simulink library "pneAux_rebuild_generic_std"  (R2016a)
settings: Solver=VariableStepAuto  StartTime=0.0  StopTime=10.0  RelTol=1e-3
undefined symbols (not defined in the file): sMP
(part 2 of 2)

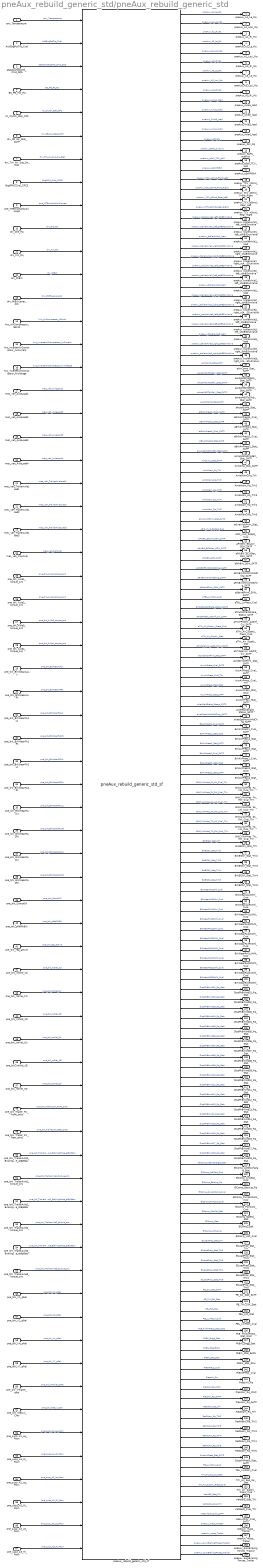
== system pneAux_rebuild_generic_std/pneAux_rebuild_generic_std ==
  env_Temperature : Inport
  ActlEngPctTrq_Cval : Inport  Port=2
  aSatpAutoOpMd_Cmd_SDS : Inport  Port=3
  BS_PB_Fct_Rq : Inport  Port=4
  ch_Clutch_Stat_CPC : Inport  Port=5
  drv_PB_Sw_Stat_SATP : Inport  Port=6
  drv_Trlr_Air_Sup_Sw_Stat : Inport  Port=7
  EngRPM_Cval_CPC3 : Inport  Port=8
  pne_MTBmodusSwAllowed : Inport  Port=9
  drv_DrS_Rq : Inport  Port=10
  drv_Knl_Rq : Inport  Port=11
  drv_PkBrk : Inport  Port=12
  drv_PkBrkLever_pos : Inport  Port=13
  hvs_AirCompressor_nEmot : Inport  Port=14
  hvs_InverterAirCompressor_hvCurrent : Inport  Port=15
  hvs_InverterAirCompressor_hvVoltage : Inport  Port=16
  mec_veh_AxleLoad1 : Inport  Port=17
  mec_veh_AxleLoad2 : Inport  Port=18
  mec_veh_AxleLoad3 : Inport  Port=19
  mec_veh_AxleLoad4 : Inport  Port=20
  mec_veh_TrailerAxleLoad1 : Inport  Port=21
  mec_veh_TrailerAxleLoad2 : Inport  Port=22
  mec_veh_TrailerAxleLoad3 : Inport  Port=23
  mec_veh_transVel : Inport  Port=24
  pne_brk_Axle1_torque_sns : Inport  Port=25
  pne_brk_Axle2_torque_sns : Inport  Port=26
  pne_brk_Axle3_torque_sns : Inport  Port=27
  pne_brk_Axle4_torque_sns : Inport  Port=28
  pne_brk_BrkWearAALt : Inport  Port=29
  pne_brk_BrkWearAARt : Inport  Port=30
  pne_brk_BrkWearFA1Lt : Inport  Port=31
  pne_brk_BrkWearFA1Rt : Inport  Port=32
  pne_brk_BrkWearFA2Lt : Inport  Port=33
  pne_brk_BrkWearFA2Rt : Inport  Port=34
  pne_brk_BrkWearRA1Lt : Inport  Port=35
  pne_brk_BrkWearRA1Rt : Inport  Port=36
  pne_brk_BrkWearRA2Lt : Inport  Port=37
  pne_brk_BrkWearRA2Rt : Inport  Port=38
  pne_brk_CompON : Inport  Port=39
  pne_brk_pRelPkBrk : Inport  Port=40
  pne_brk_reg_active : Inport  Port=41
  pne_brk_rotVel_t1l : Inport  Port=42
  pne_brk_rotVel_t1r : Inport  Port=43
  pne_brk_rotVel_t2l : Inport  Port=44
  pne_brk_rotVel_t2r : Inport  Port=45
  pne_brk_rotVel_t3l : Inport  Port=46
  pne_brk_rotVel_t3r : Inport  Port=47
  pne_brk_Trailer_RV_Front_pAct : Inport  Port=48
  pne_brk_Trailer_RV_Rear_pAct : Inport  Port=49
  pne_brk_TrailerAxle1_BrakingForce_at8p5bar : Inport  Port=50
  pne_brk_TrailerAxle1_torque_sns : Inport  Port=51
  pne_brk_TrailerAxle2_BrakingForce_at8p5bar : Inport  Port=52
  pne_brk_TrailerAxle2_torque_sns : Inport  Port=53
  pne_brk_TrailerAxle3_BrakingForce_at8p5bar : Inport  Port=54
  pne_brk_TrailerAxle3_torque_sns : Inport  Port=55
  pne_brk_V1_pRel : Inport  Port=56
  pne_brk_V2_pRel : Inport  Port=57
  pne_brk_V4_pRel : Inport  Port=58
  pne_brk_V7_pRel : Inport  Port=59
  pne_brk_VTrailer_pRel : Inport  Port=60
  pne_brk_WetLvl_Cntr : Inport  Port=61
  pne_susp_A1_Le_Posn : Inport  Port=62
  pne_susp_A1_Ri_Posn : Inport  Port=63
  pne_susp_A2_Le_Posn : Inport  Port=64
  pne_susp_A2_Ri_Posn : Inport  Port=65
  pne_susp_A3_Le_Posn : Inport  Port=66
  pne_susp_A3_Ri_Posn : Inport  Port=67
  pneAux_rebuild_generic_std_sf : S-Function  FunctionName=pneAux_rebuild_generic_std_sf  Parameters=s1 s2 p1 p2 p3 p4 p5 p6 p7 p8 p9 p10 p11 p12 p13 p14 p15 p16 p17 p18 p19 p20 p21 p22 p23 p24 p25 p26 p27 p28 p29 p30 p31 p32 p33 p34 p35 p36 p37 p38 p39 p40 p41 p42 p43 p44 p45 p46 p47 p48 p49 p50 p51 p52 p53 p54 p55 p56 p57 p58 p59 p60 p61 p62 p63 p64 p65 p66 p67 p68 p69 p70 p71 p72 p73 p74 p75 p76 p77 p78 p79 p80 p81 p82 p83 p84 p85 p86 p87 p88 p89 p90 p91 p92 p93 p94 p95 p96 p97 p98 p99 p100 p101 p102 p103 p104 p105 p106 p107 p108 p109 p110 p111 p112 p113 p114 p115 p116 p117 p118 p119 p120 p121 p122 p123 p124 p125 p126 p127 p128 p129 p130 p131 p132 p133 p134 p135 p136 p137 p138 p139 p140 p141 p142 p143 p144 p145 p146 p147 p148 p149 p150 p151 p152 p153 p154 p155 p156 p157 p158 p159 p160 p161 p162 p163 p164 p165 p166 p167 p168 p169 p170 p171 p172 p173 p174 p175 p176 p177 p178 p179 p180 p181 p182 p183 p184 p185 p186 p187 p188 p189 p190 p191 p192 p193 p194 p195 p196 p197 p198 p199 p200 p201 p202 p203 p204 p205 p206 p207 p208 p209 p210 p211 p212 p213 p214 p215 p216 p217 p218 p219 p220 p221 p222 p223 p224 p225 p226 p227 p228 p229 p230 p231 p232 p233 p234 p235 p236 p237 p238 p239 p240 p241 p242 p243 p244 p245 p246 p247 p248 p249 p250 p251 p252 p253 p254 p255 p256 p257  SFunctionModules=<binary blob, 526 chars, not shown>  SFunctionDeploymentMode=off  EnableBusSupport=off  mask{s1=s1, s2=s2, initCmd='Parameters_pneAux_rebuild_generic_std_sf', p1=p1, p2=p2, p3=p3, p4=p4, p5=p5, p6=p6, p7=p7, p8=p8, p9=p9, p10=p10, p11=p11, p12=p12, p13=p13, p14=p14, p15=p15, p16=p16, p17=p17, p18=p18, p19=p19, p20=p20, p21=p21, p22=p22, p23=p23, p24=p24, p25=p25, p26=p26, p27=p27, p28=p28, p29=p29, p30=p30, p31=p31, p32=p32, p33=p33, p34=p34, p35=p35, p36=p36, p37=p37, p38=p38, p39=p39, p40=p40, p41=p41, p42=p42, p43=p43, p44=p44, p45=p45, p46=p46, p47=p47, p48=p48, p49=p49, p50=p50, p51=p51, p52=p52, p53=p53, p54=p54, p55=p55, p56=p56, p57=p57, p58=p58, p59=p59, p60=p60, p61=p61, p62=p62, p63=p63, p64=p64, p65=p65, p66=p66, p67=p67, p68=p68, p69=p69, p70=p70, p71=p71, p72=p72, p73=p73, p74=p74, p75=p75, p76=p76, p77=p77, p78=p78, p79=p79, p80=p80, p81=p81, p82=p82, p83=p83, p84=p84, p85=p85, p86=p86, p87=p87, p88=p88, p89=p89, p90=p90, p91=p91, p92=p92, p93=p93, p94=p94, p95=p95, p96=p96, p97=p97, p98=p98, p99=p99, p100=p100, p101=p101, p102=p102, p103=p103, p104=p104, p105=p105, p106=p106, p107=p107, p108=p108, p109=p109, p110=p110, p111=p111, p112=p112, p113=p113, p114=p114, p115=p115, p116=p116, p117=p117, p118=p118, p119=p119, p120=p120, p121=p121, p122=p122, p123=p123, p124=p124, p125=p125, p126=p126, p127=p127, p128=p128, p129=p129, p130=p130, p131=p131, p132=p132, p133=p133, p134=p134, p135=p135, p136=p136, p137=p137, p138=p138, p139=p139, p140=p140, p141=p141, p142=p142, p143=p143, p144=p144, p145=p145, p146=p146, p147=p147, p148=p148, p149=p149, p150=p150, p151=p151, p152=p152, p153=p153, p154=p154, p155=p155, p156=p156, p157=p157, p158=p158, p159=p159, p160=p160, p161=p161, p162=p162, p163=p163, p164=p164, p165=p165, p166=p166, p167=p167, p168=p168, p169=p169, p170=p170, p171=p171, p172=p172, p173=p173, p174=p174, p175=p175, p176=p176, p177=p177, p178=p178, p179=p179, p180=p180, p181=p181, p182=p182, p183=p183, p184=p184, p185=p185, p186=p186, p187=p187, p188=p188, p189=p189, p190=p190, p191=p191, p192=p192, p193=p193, p194=p194, p195=p195, p196=p196, p197=p197, p198=p198, p199=p199, p200=p200, p201=p201, p202=p202, p203=p203, p204=p204, p205=p205, p206=p206, p207=p207, p208=p208, p209=p209, p210=p210, p211=p211, p212=p212, p213=p213, p214=p214, p215=p215, p216=p216, p217=p217, p218=p218, p219=p219, p220=p220, p221=p221, p222=p222, p223=p223, p224=p224, p225=p225, p226=p226, p227=p227, p228=p228, p229=p229, p230=p230, p231=p231, p232=p232, p233=p233, p234=p234, p235=p235, p236=p236, p237=p237, p238=p238, p239=p239, p240=p240, p241=p241, p242=p242, p243=p243, p244=p244, p245=p245, p246=p246, p247=p247, p248=p248, p249=p249, p250=p250, p251=p251, p252=p252, p253=p253, p254=p254, p255=p255, p256=p256, p257=p257}
      mask prompts: s1 "Solver Type: settings_iMode [-]"; s2 "Solver Step Size: settings_dt [s]"; initCmd "Initialization command"; p1 "aAirComp_Stat_SATP, Compressor status: 0,1,2,3 / inactiv, active, err, SNA export=true name=aAirComp_Stat_SATP prio=1 dataSetName=std dataClassType=initIO dataClassName=initIO unit='-' description='Compressor status: 0,1,2,3 / inactiv, active, err, SNA': pneAux.aAirComp_Stat_SATP_0 [-]"; p2 "aAutoMd1To2Rdy_Stat_SATP, L4 - Driver mode: 0,1,2,3 / not ready, ready, reserved, SNA ((ATG) Readiness status of SATP to transition from mode 1 to mode 2) export=true name=aAutoMd1To2Rdy_Stat_SATP prio=1 dataSetName=std dataClassType=initIO dataClassName=initIO unit='-' description='L4 - Driver mode: 0,1,2,3 / not ready, ready, reserved, SNA ((ATG) Readiness status of SATP to transition from mode 1 to mode 2)': pneAux.aAutoMd1To2Rdy_Stat_SATP_0 [-]"; p3 "aAutoMd1To3Rdy_Stat_SATP, L4 - Driver mode: 0,1,2,3 / not ready, ready, reserved, SNA ((ATG) Readiness status of SATP to transition from mode 1 to mode 3) export=true name=aAutoMd1To3Rdy_Stat_SATP prio=1 dataSetName=std dataClassType=initIO dataClassName=initIO unit='-' description='L4 - Driver mode: 0,1,2,3 / not ready, ready, reserved, SNA ((ATG) Readiness status of SATP to transition from mode 1 to mode 3)': pneAux.aAutoMd1To3Rdy_Stat_SATP_0 [-]"; p4 "aAutoMd3To1Rdy_Stat_SATP, L4 - Driver mode: 0,1,2,3 / not ready, ready, reserved, SNA ((ATG) Readiness status of SATP to transition from mode 3 to mode 1) export=true name=aAutoMd3To1Rdy_Stat_SATP prio=1 dataSetName=std dataClassType=initIO dataClassName=initIO unit='-' description='L4 - Driver mode: 0,1,2,3 / not ready, ready, reserved, SNA ((ATG) Readiness status of SATP to transition from mode 3 to mode 1)': pneAux.aAutoMd3To1Rdy_Stat_SATP_0 [-]"; p5 "aAutoOpMd_Stat_SATP, 0,1,2,3 /  MODE_1 Manual Mode, L4_IFTD SAE L4 with IFTD, L4_NDC SAE L4 with no driver controls, SNA Signal not Available export=true name=aAutoOpMd_Stat_SATP prio=1 dataSetName=std dataClassType=initIO dataClassName=initIO unit='-' description='0,1,2,3 /  MODE_1 Manual Mode, L4_IFTD SAE L4 with IFTD, L4_NDC SAE L4 with no driver controls, SNA Signal not Available': pneAux.aAutoOpMd_Stat_SATP_0 [-]"; p6 "aBrkAirPress1_Cval_SATP (init) export=true name=aBrkAirPress1_Cval_SATP prio=1 dataSetName=std dataClassType=initIO dataClassName=initIO unit=kPa description='aBrkAirPress1_Cval_SATP': pneAux.aBrkAirPress1_Cval_SATP_0 [-]"; p7 "aBrkAirPress1_Stat_SATP (init) export=true name=aBrkAirPress1_Stat_SATP prio=1 dataSetName=std dataClassType=initIO dataClassName=initIO unit=kPa description='aBrkAirPress1_Stat_SATP': pneAux.aBrkAirPress1_Stat_SATP_0 [-]"; p8 "aBrkAirPress2_Cval_SATP (init) export=true name=aBrkAirPress2_Cval_SATP prio=1 dataSetName=std dataClassType=initIO dataClassName=initIO unit=kPa description='aBrkAirPress2_Cval_SATP': pneAux.aBrkAirPress2_Cval_SATP_0 [-]"; p9 "aBrkAirPress2_Stat_SATP (init) export=true name=aBrkAirPress2_Stat_SATP prio=1 dataSetName=std dataClassType=initIO dataClassName=initIO unit=kPa description='aBrkAirPress2_Stat_SATP': pneAux.aBrkAirPress2_Stat_SATP_0 [-]"; p10 "ActlEngPctTrq_Cval (init) export=true name=ActlEngPctTrq_Cval prio=1 dataSetName=std dataClassType=initIO dataClassName=initIO unit='-' description='ActlEngPctTrq_Cval': pneAux.ActlEngPctTrq_Cval_0 [-]"; p11 "aImplsblMdCmdErr_Stat_SATP, 0,1,2,3 /  OK, invalid, reserved, SNA export=true name=aImplsblMdCmdErr_Stat_SATP prio=1 dataSetName=std dataClassType=initIO dataClassName=initIO unit='-' description='0,1,2,3 /  OK, invalid, reserved, SNA': pneAux.aImplsblMdCmdErr_Stat_SATP_0 [-]"; p12 "AirComp_Stat_SATP, Compressor status: 0,1,2,3 / inactiv, active, err, SNA export=true name=AirComp_Stat_SATP prio=1 dataSetName=std dataClassType=initIO dataClassName=initIO unit='-' description='Compressor status: 0,1,2,3 / inactiv, active, err, SNA': pneAux.AirComp_Stat_SATP_0 [-]"; p13 "AmbWarn_Rq_Trlr2,   export=true name=AmbWarn_Rq_Trlr2 prio=1 dataSetName=std dataClassType=initIO dataClassName=initIO unit='-' description=' ': pneAux.AmbWarn_Rq_Trlr2_0 [-]"; p14 "AmbWarn_Rq_Trlr3,   export=true name=AmbWarn_Rq_Trlr3 prio=1 dataSetName=std dataClassType=initIO dataClassName=initIO unit='-' description=' ': pneAux.AmbWarn_Rq_Trlr3_0 [-]"; p15 "AmbWarn_Rq_Trlr4,   export=true name=AmbWarn_Rq_Trlr4 prio=1 dataSetName=std dataClassType=initIO dataClassName=initIO unit='-' description=' ': pneAux.AmbWarn_Rq_Trlr4_0 [-]"; p16 "AmbWarn_Rq_Trlr5,   export=true name=AmbWarn_Rq_Trlr5 prio=1 dataSetName=std dataClassType=initIO dataClassName=initIO unit='-' description=' ': pneAux.AmbWarn_Rq_Trlr5_0 [-]"; p17 "AmbWarn_Rq_Trlr export=true name=AmbWarn_Rq_Trlr prio=1 dataSetName=std dataClassType=initIO dataClassName=initIO unit='-' description='AmbWarn_Rq_Trlr': pneAux.AmbWarn_Rq_Trlr_0 [-]"; p18 "aOverVoltPrim_Stat_SATP, 0,1,2,3 /  OK, overvoltage, reserved, SNA export=true name=aOverVoltPrim_Stat_SATP prio=1 dataSetName=std dataClassType=initIO dataClassName=initIO unit='-' description='0,1,2,3 /  OK, overvoltage, reserved, SNA': pneAux.aOverVoltPrim_Stat_SATP_0 [-]"; p19 "Inverter 2 Requested Speed API2 for air compressor (init) export=true name=API2_Inv2_RqSpd_Cval prio=1 dataSetName=std dataClassType=initIO dataClassName=initIO unit='-' description='Inverter 2 Requested Speed API2 for air compressor (init)': pneAux.API2_Inv2_RqSpd_Cval_0 [-]"; p20 "aPrkBrk_ECUAir_SOH_SATP,  (ATG) ECU  Air management health status: 0 Fully Operational / 1 Partly Operational / 2 Not Operational / 3 SNA export=true name=aPrkBrk_ECUAir_SOH_SATP prio=1 dataSetName=std dataClassType=initIO dataClassName=initIO unit='-' description=' (ATG) ECU  Air management health status: 0 Fully Operational / 1 Partly Operational / 2 Not Operational / 3 SNA': pneAux.aPrkBrk_ECUAir_SOH_SATP_0 [-]"; p21 "aPrkBrk_ECUGen_SOH_SATP,  (ATG) ECU general health status: 0 Fully Operational / 1 Partly Operational / 2 Not Operational / 3 SNA export=true name=aPrkBrk_ECUGen_SOH_SATP prio=1 dataSetName=std dataClassType=initIO dataClassName=initIO unit='-' description=' (ATG) ECU general health status: 0 Fully Operational / 1 Partly Operational / 2 Not Operational / 3 SNA': pneAux.aPrkBrk_ECUGen_SOH_SATP_0 [-]"; p22 "aPrkBrk_SOH_SATP,  (ATG) Parking Brake System Health Status: 0 Fully Operational / 1 Partly Operational / 2 Not Operational / 3 SNA export=true name=aPrkBrk_SOH_SATP prio=1 dataSetName=std dataClassType=initIO dataClassName=initIO unit='-' description=' (ATG) Parking Brake System Health Status: 0 Fully Operational / 1 Partly Operational / 2 Not Operational / 3 SNA': pneAux.aPrkBrk_SOH_SATP_0 [-]"; p23 "aPrkBrkFltIntrlckMdChng_SATP, 0,1,2,3 /  NoT met, met, reserved, SNA ((ATG) Current status in SATP for the Fault interlock for mode change) export=true name=aPrkBrkFltIntrlckMdChng_SATP prio=1 dataSetName=std dataClassType=initIO dataClassName=initIO unit='-' description='0,1,2,3 /  NoT met, met, reserved, SNA ((ATG) Current status in SATP for the Fault interlock for mode change)': pneAux.aPrkBrkFltIntrlckMdChng_SATP_0 [-]"; p24 "aPrkBrkIntrlckMdChng_SATP, 0,1,2,3 /  NoT met, met, reserved, SNA ((ATG) Current status in SATP for the park brake interlock for mode change) export=true name=aPrkBrkIntrlckMdChng_SATP prio=1 dataSetName=std dataClassType=initIO dataClassName=initIO unit='-' description='0,1,2,3 /  NoT met, met, reserved, SNA ((ATG) Current status in SATP for the park brake interlock for mode change)': pneAux.aPrkBrkIntrlckMdChng_SATP_0 [-]"; p25 "aSatpAutoOpMd_Cmd_SDS (init) export=true name=aSatpAutoOpMd_Cmd_SDS prio=1 dataSetName=std dataClassType=initIO dataClassName=initIO unit='-' description='SATP operational mode command by SDS': pneAux.aSatpAutoOpMd_Cmd_SDS_0 [-]"; p26 "aSdsIntfPrim_SOH_SATP,   export=true name=aSdsIntfPrim_SOH_SATP prio=1 dataSetName=std dataClassType=initIO dataClassName=initIO unit='-' description=' ': pneAux.aSdsIntfPrim_SOH_SATP_0 [-]"; p27 "aTBL_LvrPosn_Cval, Lever: 0..100, 101..253,254,255 / 0..100, RES,ERR,SNA export=true name=aTBL_LvrPosn_Cval prio=1 dataSetName=std dataClassType=initIO dataClassName=initIO unit='%' description='Lever: 0..100, 101..253,254,255 / 0..100, RES,ERR,SNA': pneAux.aTBL_LvrPosn_Cval_0 [-]"; p28 "ATBVehicleParameter (0-disabled, 1-enabled) export=true name=ATBVehicleParameter prio=1 dataSetName=pneAux_dummy dataClassType=main dataClassName=main unit='-' description='ATBVehicleParameter (0-disabled, 1-enabled)': pneAux.ATBVehicleParameter [-]"; p29 "aTractorParkBrake_Status_SATP, 0,1,2,6,7 / ENGG Engaged, INT Intermediate Position, DISENGG Disengaged, ERR, SNA ((ATG)  export=true name=aTractorParkBrake_Status_SATP prio=1 dataSetName=std dataClassType=initIO dataClassName=initIO unit='-' description='0,1,2,6,7 / ENGG Engaged, INT Intermediate Position, DISENGG Disengaged, ERR, SNA ((ATG) ': pneAux.aTractorParkBrake_Status_SATP_0 [-]"; p30 "aTrctrPrkBrk_AddInf_Cvl_SATP, 0,1,2,6,7 / DEFLATED Deflated (parked), INT Intermediate, INFLATED Inflated (unparked), ERR, SNA ((ATG)  export=true name=aTrctrPrkBrk_AddInf_Cvl_SATP prio=1 dataSetName=std dataClassType=initIO dataClassName=initIO unit='-' description='0,1,2,6,7 / DEFLATED Deflated (parked), INT Intermediate, INFLATED Inflated (unparked), ERR, SNA ((ATG) ': pneAux.aTrctrPrkBrk_AddInf_Cvl_SATP_0 [-]"; p31 "aTrlr_Air_Supply_Press_Cval, 0..250,251..253,254,255 / 0..2000, RES,ERR,SNA export=true name=aTrlr_Air_Supply_Press_Cval prio=1 dataSetName=std dataClassType=initIO dataClassName=initIO unit='kPa' description='0..250,251..253,254,255 / 0..2000, RES,ERR,SNA': pneAux.aTrlr_Air_Supply_Press_Cval_0 [-]"; p32 "aTrlr_Air_Supply_Stat (init), 0,1,2,3 / SPL supplied, NSPL not supplied, ERR, SAN ((ATG) Trailer Air Supply Current state) export=true name=aTrlr_Air_Supply_Stat prio=1 dataSetName=std dataClassType=initIO dataClassName=initIO unit='-' description='0,1,2,3 / SPL supplied, NSPL not supplied, ERR, SAN ((ATG) Trailer Air Supply Current state)': pneAux.aTrlr_Air_Supply_Stat_0 [-]"; p33 "aTrlrSpplyLn_AddInf_Cvl_SATP, 0,1,2,3 / HIGH_INT Signal integrity High, 1 LOW_INT Signal Integrity low, 2 NO_SENSING no sensing possible, SNA ((ATG) Trailer Supply Line Additional  export=true name=aTrlrSpplyLn_AddInf_Cvl_SATP prio=1 dataSetName=std dataClassType=initIO dataClassName=initIO unit='-' description='0,1,2,3 / HIGH_INT Signal integrity High, 1 LOW_INT Signal Integrity low, 2 NO_SENSING no sensing possible, SNA ((ATG) Trailer Supply Line Additional ': pneAux.aTrlrSpplyLn_AddInf_Cvl_SATP_0 [-]"; p34 "aUnderVoltPrim_Stat_SATP, (ATG) Primary Under Voltage Status SBSP export=true name=aUnderVoltPrim_Stat_SATP prio=1 dataSetName=std dataClassType=initIO dataClassName=initIO unit='-' description='(ATG) Primary Under Voltage Status SBSP': pneAux.aUnderVoltPrim_Stat_SATP_0 [-]"; p35 "AuxAirPress_Cval_SATP (init) export=true name=AuxAirPress_Cval_SATP prio=1 dataSetName=std dataClassType=initIO dataClassName=initIO unit=kPa description='AuxAirPress_Cval_SATP': pneAux.AuxAirPress_Cval_SATP_0 [-]"; p36 "AuxAirPress_Cval_Trlr (init) export=true name=AuxAirPress_Cval_Trlr prio=1 dataSetName=std dataClassType=initIO dataClassName=initIO unit=kPa description='AuxAirPress_Cval_Trlr': pneAux.AuxAirPress_Cval_Trlr_0 [-]"; p37 "AuxAirPress_Stat_ICUC (init) export=true name=AuxAirPress_Stat_ICUC prio=1 dataSetName=std dataClassType=initIO dataClassName=initIO unit=kPa description='AuxAirPress_Stat_ICUC': pneAux.AuxAirPress_Stat_ICUC_0 [-]"; p38 "AuxAirPress_Stat_SATP (init) export=true name=AuxAirPress_Stat_SATP prio=1 dataSetName=std dataClassType=initIO dataClassName=initIO unit=kPa description='AuxAirPress_Stat_SATP': pneAux.AuxAirPress_Stat_SATP_0 [-]"; p39 "aVehParkBrake_Status_SATP, Parking Brake Status entire vehicle: 0,1,2,3,6,7 / SAFE_PARK Safety Parked, NO_DRIVEOFF Drive-Off Inhibited, SAFE_DRIVEOFF_CBN Safe Drive-Off Combined, SAFE_DRIVEOFF_BT Safe Drive-Off- Bobtail, ERR, SNA ((ATG)  export=true name=aVehParkBrake_Status_SATP prio=1 dataSetName=std dataClassType=initIO dataClassName=initIO unit='-' description='Parking Brake Status entire vehicle: 0,1,2,3,6,7 / SAFE_PARK Safety Parked, NO_DRIVEOFF Drive-Off Inhibited, SAFE_DRIVEOFF_CBN Safe Drive-Off Combined, SAFE_DRIVEOFF_BT Safe Drive-Off- Bobtail, ERR, SNA ((ATG) ': pneAux.aVehParkBrake_Status_SATP_0 [-]"; p40 "aVehSpdIntrlckMdChng_SATP, 0,1,2,3 / NoT met, met, reserved, SNA ((ATG) Current status in SATP for the vehicle speed interlock for mode change export=true name=aVehSpdIntrlckMdChng_SATP prio=1 dataSetName=std dataClassType=initIO dataClassName=initIO unit='-' description='0,1,2,3 / NoT met, met, reserved, SNA ((ATG) Current status in SATP for the vehicle speed interlock for mode change': pneAux.aVehSpdIntrlckMdChng_SATP_0 [-]"; p41 "BrkAirPress1_Cval_SATP (init) export=true name=BrkAirPress1_Cval_SATP prio=1 dataSetName=std dataClassType=initIO dataClassName=initIO unit=kPa description='BrkAirPress1_Cval_SATP': pneAux.BrkAirPress1_Cval_SATP_0 [-]"; p42 "BrkAirPress1_Stat_ICUC (init) export=true name=BrkAirPress1_Stat_ICUC prio=1 dataSetName=std dataClassType=initIO dataClassName=initIO unit=kPa description='BrkAirPress1_Stat_ICUC': pneAux.BrkAirPress1_Stat_ICUC_0 [-]"; p43 "BrkAirPress1_Stat_SATP (init) export=true name=BrkAirPress1_Stat_SATP prio=1 dataSetName=std dataClassType=initIO dataClassName=initIO unit=kPa description='BrkAirPress1_Stat_SATP': pneAux.BrkAirPress1_Stat_SATP_0 [-]"; p44 "BrkAirPress2_Cval_SATP (init) export=true name=BrkAirPress2_Cval_SATP prio=1 dataSetName=std dataClassType=initIO dataClassName=initIO unit=kPa description='BrkAirPress2_Cval_SATP': pneAux.BrkAirPress2_Cval_SATP_0 [-]"; p45 "BrkAirPress2_Stat_ICUC (init) export=true name=BrkAirPress2_Stat_ICUC prio=1 dataSetName=std dataClassType=initIO dataClassName=initIO unit=kPa description='BrkAirPress2_Stat_ICUC': pneAux.BrkAirPress2_Stat_ICUC_0 [-]"; p46 "BrkAirPress2_Stat_SATP (init) export=true name=BrkAirPress2_Stat_SATP prio=1 dataSetName=std dataClassType=initIO dataClassName=initIO unit=kPa description='BrkAirPress2_Stat_SATP': pneAux.BrkAirPress2_Stat_SATP_0 [-]"; p47 "Trailer brake pressur first axle left wheel (init) export=true name=BrkCylAirPres_FA_LW_Cval_Trlr prio=1 dataSetName=std dataClassType=initIO dataClassName=initIO unit=kPa description='Trailer brake pressur first axle left wheel': pneAux.BrkCylAirPres_FA_LW_Cval_Trlr_0 [-]"; p48 "Trailer brake pressur first axle right wheel (init) export=true name=BrkCylAirPres_FA_RW_Cval_Trlr prio=1 dataSetName=std dataClassType=initIO dataClassName=initIO unit=kPa description='Trailer brake pressur first axle right wheel': pneAux.BrkCylAirPres_FA_RW_Cval_Trlr_0 [-]"; p49 "Trailer brake pressur second axle left wheel (init) export=true name=BrkCylAirPres_SA_LW_Cval_Trlr prio=1 dataSetName=std dataClassType=initIO dataClassName=initIO unit=kPa description='Trailer brake pressur second axle left wheel': pneAux.BrkCylAirPres_SA_LW_Cval_Trlr_0 [-]"; p50 "Trailer brake pressur second axle right wheel (init) export=true name=BrkCylAirPres_SA_RW_Cval_Trlr prio=1 dataSetName=std dataClassType=initIO dataClassName=initIO unit=kPa description='Trailer brake pressur second axle right wheel': pneAux.BrkCylAirPres_SA_RW_Cval_Trlr_0 [-]"; p51 "Trailer brake pressur third axle left wheel (init) export=true name=BrkCylAirPres_TA_LW_Cval_Trlr prio=1 dataSetName=std dataClassType=initIO dataClassName=initIO unit=kPa description='Trailer brake pressur third axle left wheel': pneAux.BrkCylAirPres_TA_LW_Cval_Trlr_0 [-]"; p52 "Trailer brake pressur third axle right wheel (init) export=true name=BrkCylAirPres_TA_RW_Cval_Trlr prio=1 dataSetName=std dataClassType=initIO dataClassName=initIO unit=kPa description='Trailer brake pressur third axle right wheel': pneAux.BrkCylAirPres_TA_RW_Cval_Trlr_0 [-]"; p53 "BrkElCtrl_Stat_Trlr2,   export=true name=BrkElCtrl_Stat_Trlr2 prio=1 dataSetName=std dataClassType=initIO dataClassName=initIO unit='-' description=' ': pneAux.BrkElCtrl_Stat_Trlr2_0 [-]"; p54 "BrkElCtrl_Stat_Trlr3,   export=true name=BrkElCtrl_Stat_Trlr3 prio=1 dataSetName=std dataClassType=initIO dataClassName=initIO unit='-' description=' ': pneAux.BrkElCtrl_Stat_Trlr3_0 [-]"; p55 "BrkElCtrl_Stat_Trlr4,   export=true name=BrkElCtrl_Stat_Trlr4 prio=1 dataSetName=std dataClassType=initIO dataClassName=initIO unit='-' description=' ': pneAux.BrkElCtrl_Stat_Trlr4_0 [-]"; p56 "BrkElCtrl_Stat_Trlr5,   export=true name=BrkElCtrl_Stat_Trlr5 prio=1 dataSetName=std dataClassType=initIO dataClassName=initIO unit='-' description=' ': pneAux.BrkElCtrl_Stat_Trlr5_0 [-]"; p57 "BrkElCtrl_Stat_Trlr export=true name=BrkElCtrl_Stat_Trlr prio=1 dataSetName=std dataClassType=initIO dataClassName=initIO unit='-' description='BrkElCtrl_Stat_Trlr': pneAux.BrkElCtrl_Stat_Trlr_0 [-]"; p58 "BrkWearAALtWhl_Cval export=true name=BrkWearAALtWhl_Cval prio=1 dataSetName=std dataClassType=initIO dataClassName=initIO unit='%' description='BrkWearAALtWhl_Cval': pneAux.BrkWearAALtWhl_Cval_0 [-]"; p59 "BrkWearAARtWhl_Cval export=true name=BrkWearAARtWhl_Cval prio=1 dataSetName=std dataClassType=initIO dataClassName=initIO unit='%' description='BrkWearAARtWhl_Cval': pneAux.BrkWearAARtWhl_Cval_0 [-]"; p60 "BrkWearFA1LtWhl_Cval export=true name=BrkWearFA1LtWhl_Cval prio=1 dataSetName=std dataClassType=initIO dataClassName=initIO unit='%' description='BrkWearFA1LtWhl_Cval': pneAux.BrkWearFA1LtWhl_Cval_0 [-]"; p61 "BrkWearFA1LtWhl_Cval export=true name=BrkWearFA1RtWhl_Cval prio=1 dataSetName=std dataClassType=initIO dataClassName=initIO unit='%' description='BrkWearFA1RtWhl_Cval': pneAux.BrkWearFA1RtWhl_Cval_0 [-]"; p62 "BrkWearFA1LtWhl_Cval export=true name=BrkWearFA2LtWhl_Cval prio=1 dataSetName=std dataClassType=initIO dataClassName=initIO unit='%' description='BrkWearFA2LtWhl_Cval': pneAux.BrkWearFA2LtWhl_Cval_0 [-]"; p63 "BrkWearFA1LtWhl_Cval export=true name=BrkWearFA2RtWhl_Cval prio=1 dataSetName=std dataClassType=initIO dataClassName=initIO unit='%' description='BrkWearFA2RtWhl_Cval': pneAux.BrkWearFA2RtWhl_Cval_0 [-]"; p64 "BrkWearRA1LtWhl_Cval export=true name=BrkWearRA1LtWhl_Cval prio=1 dataSetName=std dataClassType=initIO dataClassName=initIO unit='%' description='BrkWearRA1LtWhl_Cval': pneAux.BrkWearRA1LtWhl_Cval_0 [-]"; p65 "BrkWearRA1LtWhl_Cval export=true name=BrkWearRA1RtWhl_Cval prio=1 dataSetName=std dataClassType=initIO dataClassName=initIO unit='%' description='BrkWearRA1RtWhl_Cval': pneAux.BrkWearRA1RtWhl_Cval_0 [-]"; p66 "BrkWearRA1LtWhl_Cval export=true name=BrkWearRA2LtWhl_Cval prio=1 dataSetName=std dataClassType=initIO dataClassName=initIO unit='%' description='BrkWearRA2LtWhl_Cval': pneAux.BrkWearRA2LtWhl_Cval_0 [-]"; p67 "BrkWearRA1LtWhl_Cval export=true name=BrkWearRA2RtWhl_Cval prio=1 dataSetName=std dataClassType=initIO dataClassName=initIO unit='%' description='BrkWearRA2RtWhl_Cval': pneAux.BrkWearRA2RtWhl_Cval_0 [-]"; p68 "BS_PB_Fct_Rq (init) export=true name=BS_PB_Fct_Rq prio=1 dataSetName=std dataClassType=initIO dataClassName=initIO unit='-' description='BS_PB_Fct_Rq': pneAux.BS_PB_Fct_Rq_0 [-]"; p69 "ch_Clutch_Stat_CPC (init) export=true name=ch_Clutch_Stat_CPC prio=1 dataSetName=std dataClassType=initIO dataClassName=initIO unit='-' description='ch_Clutch_Stat_CPC (init)': pneAux.ch_Clutch_Stat_CPC_0 [-]"; p70 "DispPkBrkInd01_Rq_Stat, 0,1,2,3 / not requested, requested, res, sna (Display Park(ing) Brake(ing) Indication/Indicator 01 Requested state Current state export=true name=DispPkBrkInd01_Rq_Stat prio=1 dataSetName=std dataClassType=initIO dataClassName=initIO unit='-' description='0,1,2,3 / not requested, requested, res, sna (Display Park(ing) Brake(ing) Indication/Indicator 01 Requested state Current state': pneAux.DispPkBrkInd01_Rq_Stat_0 [-]"; p71 "DispPkBrkInd02_Rq_Stat, 0,1,2,3 / not requested, requested, res, sna (Display Park(ing) Brake(ing) Indication/Indicator 01 Requested state Current state export=true name=DispPkBrkInd02_Rq_Stat prio=1 dataSetName=std dataClassType=initIO dataClassName=initIO unit='-' description='0,1,2,3 / not requested, requested, res, sna (Display Park(ing) Brake(ing) Indication/Indicator 01 Requested state Current state': pneAux.DispPkBrkInd02_Rq_Stat_0 [-]"; p72 "DispPkBrkInd03_Rq_Stat, 0,1,2,3 / not requested, requested, res, sna (Display Park(ing) Brake(ing) Indication/Indicator 01 Requested state Current state export=true name=DispPkBrkInd03_Rq_Stat prio=1 dataSetName=std dataClassType=initIO dataClassName=initIO unit='-' description='0,1,2,3 / not requested, requested, res, sna (Display Park(ing) Brake(ing) Indication/Indicator 01 Requested state Current state': pneAux.DispPkBrkInd03_Rq_Stat_0 [-]"; p73 "DispPkBrkInd04_Rq_Stat, 0,1,2,3 / not requested, requested, res, sna (Display Park(ing) Brake(ing) Indication/Indicator 01 Requested state Current state export=true name=DispPkBrkInd04_Rq_Stat prio=1 dataSetName=std dataClassType=initIO dataClassName=initIO unit='-' description='0,1,2,3 / not requested, requested, res, sna (Display Park(ing) Brake(ing) Indication/Indicator 01 Requested state Current state': pneAux.DispPkBrkInd04_Rq_Stat_0 [-]"; p74 "DispPkBrkInd05_Rq_Stat, 0,1,2,3 / not requested, requested, res, sna (Display Park(ing) Brake(ing) Indication/Indicator 01 Requested state Current state export=true name=DispPkBrkInd05_Rq_Stat prio=1 dataSetName=std dataClassType=initIO dataClassName=initIO unit='-' description='0,1,2,3 / not requested, requested, res, sna (Display Park(ing) Brake(ing) Indication/Indicator 01 Requested state Current state': pneAux.DispPkBrkInd05_Rq_Stat_0 [-]"; p75 "DispPkBrkInd06_Rq_Stat, 0,1,2,3 / not requested, requested, res, sna (Display Park(ing) Brake(ing) Indication/Indicator 01 Requested state Current state export=true name=DispPkBrkInd06_Rq_Stat prio=1 dataSetName=std dataClassType=initIO dataClassName=initIO unit='-' description='0,1,2,3 / not requested, requested, res, sna (Display Park(ing) Brake(ing) Indication/Indicator 01 Requested state Current state': pneAux.DispPkBrkInd06_Rq_Stat_0 [-]"; p76 "DispPkBrkInd07_Rq_Stat, 0,1,2,3 / not requested, requested, res, sna (Display Park(ing) Brake(ing) Indication/Indicator 01 Requested state Current state export=true name=DispPkBrkInd07_Rq_Stat prio=1 dataSetName=std dataClassType=initIO dataClassName=initIO unit='-' description='0,1,2,3 / not requested, requested, res, sna (Display Park(ing) Brake(ing) Indication/Indicator 01 Requested state Current state': pneAux.DispPkBrkInd07_Rq_Stat_0 [-]"; p77 "DispPkBrkInd08_Rq_Stat, 0,1,2,3 / not requested, requested, res, sna (Display Park(ing) Brake(ing) Indication/Indicator 01 Requested state Current state export=true name=DispPkBrkInd08_Rq_Stat prio=1 dataSetName=std dataClassType=initIO dataClassName=initIO unit='-' description='0,1,2,3 / not requested, requested, res, sna (Display Park(ing) Brake(ing) Indication/Indicator 01 Requested state Current state': pneAux.DispPkBrkInd08_Rq_Stat_0 [-]"; p78 "DispPkBrkInd09_Rq_Stat, 0,1,2,3 / not requested, requested, res, sna (Display Park(ing) Brake(ing) Indication/Indicator 01 Requested state Current state export=true name=DispPkBrkInd09_Rq_Stat prio=1 dataSetName=std dataClassType=initIO dataClassName=initIO unit='-' description='0,1,2,3 / not requested, requested, res, sna (Display Park(ing) Brake(ing) Indication/Indicator 01 Requested state Current state': pneAux.DispPkBrkInd09_Rq_Stat_0 [-]"; p79 "DispPkBrkInd10_Rq_Stat, 0,1,2,3 / not requested, requested, res, sna (Display Park(ing) Brake(ing) Indication/Indicator 01 Requested state Current state export=true name=DispPkBrkInd10_Rq_Stat prio=1 dataSetName=std dataClassType=initIO dataClassName=initIO unit='-' description='0,1,2,3 / not requested, requested, res, sna (Display Park(ing) Brake(ing) Indication/Indicator 01 Requested state Current state': pneAux.DispPkBrkInd10_Rq_Stat_0 [-]"; p80 "DispPkBrkInd11_Rq_Stat, 0,1,2,3 / not requested, requested, res, sna (Display Park(ing) Brake(ing) Indication/Indicator 01 Requested state Current state export=true name=DispPkBrkInd11_Rq_Stat prio=1 dataSetName=std dataClassType=initIO dataClassName=initIO unit='-' description='0,1,2,3 / not requested, requested, res, sna (Display Park(ing) Brake(ing) Indication/Indicator 01 Requested state Current state': pneAux.DispPkBrkInd11_Rq_Stat_0 [-]"; p81 "DispPkBrkInd12_Rq_Stat, 0,1,2,3 / not requested, requested, res, sna (Display Park(ing) Brake(ing) Indication/Indicator 01 Requested state Current state export=true name=DispPkBrkInd12_Rq_Stat prio=1 dataSetName=std dataClassType=initIO dataClassName=initIO unit='-' description='0,1,2,3 / not requested, requested, res, sna (Display Park(ing) Brake(ing) Indication/Indicator 01 Requested state Current state': pneAux.DispPkBrkInd12_Rq_Stat_0 [-]"; p82 "DispPkBrkInd13_Rq_Stat, 0,1,2,3 / not requested, requested, res, sna (Display Park(ing) Brake(ing) Indication/Indicator 01 Requested state Current state export=true name=DispPkBrkInd13_Rq_Stat prio=1 dataSetName=std dataClassType=initIO dataClassName=initIO unit='-' description='0,1,2,3 / not requested, requested, res, sna (Display Park(ing) Brake(ing) Indication/Indicator 01 Requested state Current state': pneAux.DispPkBrkInd13_Rq_Stat_0 [-]"; p83 "DispPkBrkInd14_Rq_Stat, 0,1,2,3 / not requested, requested, res, sna (Display Park(ing) Brake(ing) Indication/Indicator 01 Requested state Current state export=true name=DispPkBrkInd14_Rq_Stat prio=1 dataSetName=std dataClassType=initIO dataClassName=initIO unit='-' description='0,1,2,3 / not requested, requested, res, sna (Display Park(ing) Brake(ing) Indication/Indicator 01 Requested state Current state': pneAux.DispPkBrkInd14_Rq_Stat_0 [-]"; p84 "DispPkBrkInd15_Rq_Stat, 0,1,2,3 / not requested, requested, res, sna (Display Park(ing) Brake(ing) Indication/Indicator 01 Requested state Current state export=true name=DispPkBrkInd15_Rq_Stat prio=1 dataSetName=std dataClassType=initIO dataClassName=initIO unit='-' description='0,1,2,3 / not requested, requested, res, sna (Display Park(ing) Brake(ing) Indication/Indicator 01 Requested state Current state': pneAux.DispPkBrkInd15_Rq_Stat_0 [-]"; p85 "DispPkBrkInd16_Rq_Stat, 0,1,2,3 / not requested, requested, res, sna (Display Park(ing) Brake(ing) Indication/Indicator 01 Requested state Current state export=true name=DispPkBrkInd16_Rq_Stat prio=1 dataSetName=std dataClassType=initIO dataClassName=initIO unit='-' description='0,1,2,3 / not requested, requested, res, sna (Display Park(ing) Brake(ing) Indication/Indicator 01 Requested state Current state': pneAux.DispPkBrkInd16_Rq_Stat_0 [-]"; p86 "DispPkBrkInd17_Rq_Stat, 0,1,2,3 / not requested, requested, res, sna (Display Park(ing) Brake(ing) Indication/Indicator 01 Requested state Current state export=true name=DispPkBrkInd17_Rq_Stat prio=1 dataSetName=std dataClassType=initIO dataClassName=initIO unit='-' description='0,1,2,3 / not requested, requested, res, sna (Display Park(ing) Brake(ing) Indication/Indicator 01 Requested state Current state': pneAux.DispPkBrkInd17_Rq_Stat_0 [-]"; p87 "DispPkBrkInd18_Rq_Stat, 0,1,2,3 / not requested, requested, res, sna (Display Park(ing) Brake(ing) Indication/Indicator 01 Requested state Current state export=true name=DispPkBrkInd18_Rq_Stat prio=1 dataSetName=std dataClassType=initIO dataClassName=initIO unit='-' description='0,1,2,3 / not requested, requested, res, sna (Display Park(ing) Brake(ing) Indication/Indicator 01 Requested state Current state': pneAux.DispPkBrkInd18_Rq_Stat_0 [-]"; p88 "drv_DrS_Rq (init) export=true name=drv_DrS_Rq prio=1 dataSetName=std dataClassType=initIO dataClassName=initIO unit='-' description='drv_DrS_Rq': pneAux.drv_DrS_Rq_0 [-]"; p89 "drv_Knl_Rq (init) export=true name=drv_Knl_Rq prio=1 dataSetName=std dataClassType=initIO dataClassName=initIO unit='-' description='drv_Knl_Rq': pneAux.drv_Knl_Rq_0 [-]"; p90 "drv_PB_Sw_Stat_SATP (init) export=true name=drv_PB_Sw_Stat_SATP prio=1 dataSetName=std dataClassType=initIO dataClassName=initIO unit='-' description='Parking brake button: 0,1,2,3 / Not Pressed, Pressed, ERR, SNA)': pneAux.drv_PB_Sw_Stat_SATP_0 [-]"; p91 "drv_PkBrk (init) export=true name=drv_PkBrk prio=1 dataSetName=std dataClassType=initIO dataClassName=initIO unit='-' description='drv_PkBrk': pneAux.drv_PkBrk_0 [-]"; p92 "drv_PkBrkLever_pos (init) export=true name=drv_PkBrkLever_pos prio=1 dataSetName=std dataClassType=initIO dataClassName=initIO unit=% description='drv_PkBrkLever_pos': pneAux.drv_PkBrkLever_pos_0 [-]"; p93 "drv_Trlr_Air_Sup_Sw_Stat (init) export=true name=drv_Trlr_Air_Sup_Sw_Stat prio=1 dataSetName=std dataClassType=initIO dataClassName=initIO unit='-' description='Trailer Air Supply Switch Status for DTNA Varian: 0,1,2,3 /  Neutral, Pulled (Apply PB), Pushed (Release PB), SNA': pneAux.drv_Trlr_Air_Sup_Sw_Stat_0 [-]"; p94 "ElComp_ActDischarge_Stat, ElComp_ActDischarge_Stat  export=true name=ElComp_ActDischarge_Stat prio=1 dataSetName=std dataClassType=initIO dataClassName=initIO unit='-' description='ElComp_ActDischarge_Stat ': pneAux.ElComp_ActDischarge_Stat_0 [-]"; p95 "ElComp_ActlSpd_Cval, Compressor ON [0 - ON, 1 - OFF] export=true name=ElComp_ActlSpd_Cval prio=1 dataSetName=std dataClassType=initIO dataClassName=initIO unit='rpm' description='Compressor ON [0 - ON, 1 - OFF]': pneAux.ElComp_ActlSpd_Cval_0 [-]"; p96 "ElComp_Backup_Rq, ElComp_Backup_Rq  0,1,2,3 / not requested, requested, ERR, SNA --> disturbed communication export=true name=ElComp_Backup_Rq prio=1 dataSetName=std dataClassType=initIO dataClassName=initIO unit='-' description='ElComp_Backup_Rq  0,1,2,3 / not requested, requested, ERR, SNA --> disturbed communication': pneAux.ElComp_Backup_Rq_0 [-]"; p97 "ElComp_CurrentCons_Cval, ElComp_CurrentCons_Cval  0..50, 51..61,62,63 / 0 .. 50,RES,ERR,SNA export=true name=ElComp_CurrentCons_Cval prio=1 dataSetName=std dataClassType=initIO dataClassName=initIO unit='A' description='ElComp_CurrentCons_Cval  0..50, 51..61,62,63 / 0 .. 50,RES,ERR,SNA': pneAux.ElComp_CurrentCons_Cval_0 [-]"; p98 "ElComp_PwrCons_Cval, ElComp_PwrCons_Cval  0..250,251..253,254,255 /  0..12.5, RES,ERR,SNA (E-Compressor power consumption) export=true name=ElComp_PwrCons_Cval prio=1 dataSetName=std dataClassType=initIO dataClassName=initIO unit='kW' description='ElComp_PwrCons_Cval  0..250,251..253,254,255 /  0..12.5, RES,ERR,SNA (E-Compressor power consumption)': pneAux.ElComp_PwrCons_Cval_0 [-]"; p99 "ElComp_SpdMd_Stat, ElComp_SpdMd_Stat  0,1,2,3 / low, med, high SNA (E-compressor speed mode Current state) export=true name=ElComp_SpdMd_Stat prio=1 dataSetName=std dataClassType=initIO dataClassName=initIO unit='-' description='ElComp_SpdMd_Stat  0,1,2,3 / low, med, high SNA (E-compressor speed mode Current state)': pneAux.ElComp_SpdMd_Stat_0 [-]"; p100 "ElComp_Stat, ElComp_Stat  0,1,2,3 /  off, on err, sna (E-Compressor activation state) export=true name=ElComp_Stat prio=1 dataSetName=std dataClassType=initIO dataClassName=initIO unit='-' description='ElComp_Stat  0,1,2,3 /  off, on err, sna (E-Compressor activation state)': pneAux.ElComp_Stat_0 [-]"; p101 "ElComp_Volt_Cval, ElComp_Volt_Cval  0..250,251..253,254,255 /  0..1000, RES,ERR,SNA export=true name=ElComp_Volt_Cval prio=1 dataSetName=std dataClassType=initIO dataClassName=initIO unit='V' description='ElComp_Volt_Cval  0..250,251..253,254,255 /  0..1000, RES,ERR,SNA': pneAux.ElComp_Volt_Cval_0 [-]"; p102 "ElLoadProp_Stat_Trlr2,   export=true name=ElLoadProp_Stat_Trlr2 prio=1 dataSetName=std dataClassType=initIO dataClassName=initIO unit='-' description=' ': pneAux.ElLoadProp_Stat_Trlr2_0 [-]"; p103 "ElLoadProp_Stat_Trlr3,   export=true name=ElLoadProp_Stat_Trlr3 prio=1 dataSetName=std dataClassType=initIO dataClassName=initIO unit='-' description=' ': pneAux.ElLoadProp_Stat_Trlr3_0 [-]"; p104 "ElLoadProp_Stat_Trlr4,   export=true name=ElLoadProp_Stat_Trlr4 prio=1 dataSetName=std dataClassType=initIO dataClassName=initIO unit='-' description=' ': pneAux.ElLoadProp_Stat_Trlr4_0 [-]"; p105 "ElLoadProp_Stat_Trlr5,   export=true name=ElLoadProp_Stat_Trlr5 prio=1 dataSetName=std dataClassType=initIO dataClassName=initIO unit='-' description=' ': pneAux.ElLoadProp_Stat_Trlr5_0 [-]"; p106 "ElLoadProp_Stat_Trlr export=true name=ElLoadProp_Stat_Trlr prio=1 dataSetName=std dataClassType=initIO dataClassName=initIO unit='-' description='ElLoadProp_Stat_Trlr': pneAux.ElLoadProp_Stat_Trlr_0 [-]"; p107 "EngRPM_Cval_CPC3 (init) export=true name=EngRPM_Cval_CPC3 prio=1 dataSetName=std dataClassType=initIO dataClassName=initIO unit='-' description='EngRPM_Cval_CPC3': pneAux.EngRPM_Cval_CPC3_0 [-]"; p108 "amb air Temperature (init) export=true name=env_Temperature prio=1 dataSetName=std dataClassType=initIO dataClassName=initIO unit=degC description='env_Temperature': pneAux.env_Temperature_0 [-]"; p109 "Tolerance Band Level AirSpring +/- [mm] export=true name=epsLevel prio=1 dataSetName=pneAux_dummy dataClassType=main dataClassName=main unit='mm' description='Tolerance Level AirSpring +/- [mm]': pneAux.epsLevel [-]"; p110 "Trailer ABS Config (0 - none, 1- ABS, 2 - EBS (incl. ABS))  export=true name=flagTrailerABS prio=1 dataSetName=veh_dummy dataClassType=veh dataClassName=veh unit='' description='Trailer ABS Config (0 - none, 1- ABS, 2 - EBS (incl. ABS))': pneAux.flagTrailerABS [-]"; p111 "hvs_AirCompressor_nEmot (init) export=true name=hvs_AirCompressor_nEmot prio=1 dataSetName=std dataClassType=initIO dataClassName=initIO unit='rpm' description='Air Compressor E-Motor speed': pneAux.hvs_AirCompressor_nEmot_0 [-]"; p112 "hvs_InverterAirCompressor_hvCurrent (init) export=true name=hvs_InverterAirCompressor_hvCurrent prio=1 dataSetName=std dataClassType=initIO dataClassName=initIO unit='A' description='Air compressor inverter hv current': pneAux.hvs_InverterAirCompressor_hvCurrent_0 [-]"; p113 "hvs_InverterAirCompressor_hvVoltage (init) export=true name=hvs_InverterAirCompressor_hvVoltage prio=1 dataSetName=std dataClassType=initIO dataClassName=initIO unit='V' description='Air compressor inverter hv voltage': pneAux.hvs_InverterAirCompressor_hvVoltage_0 [-]"; p114 "kneelingLevel [mm] export=true name=kneelingLevel prio=1 dataSetName=pneAux_dummy dataClassType=main dataClassName=main unit='mm' description='kneelingLevel' : pneAux.kneelingLevel [-]"; p115 "Compressor Speed High [rpm] export=true name=LP_rpmHigh prio=1 dataSetName=pneAux_dummy dataClassType=main dataClassName=main unit='rpm' description='Compressor Speed High [rpm]': pneAux.LP_rpmHigh [-]"; p116 "Compressor Speed Low [rpm] export=true name=LP_rpmLow prio=1 dataSetName=pneAux_dummy dataClassType=main dataClassName=main unit='rpm' description='Compressor Speed Low [rpm]': pneAux.LP_rpmLow [-]"; p117 "mec_veh_AxleLoad1 (init) export=true name=mec_veh_AxleLoad1 prio=1 dataSetName=std dataClassType=initIO dataClassName=initIO unit=kg description='mec_veh_AxleLoad1': pneAux.mec_veh_AxleLoad1_0 [-]"; p118 "mec_veh_AxleLoad2 (init) export=true name=mec_veh_AxleLoad2 prio=1 dataSetName=std dataClassType=initIO dataClassName=initIO unit=kg description='mec_veh_AxleLoad2': pneAux.mec_veh_AxleLoad2_0 [-]"; p119 "mec_veh_AxleLoad3 (init) export=true name=mec_veh_AxleLoad3 prio=1 dataSetName=std dataClassType=initIO dataClassName=initIO unit=kg description='mec_veh_AxleLoad3': pneAux.mec_veh_AxleLoad3_0 [-]"; p120 "mec_veh_AxleLoad4 (init) export=true name=mec_veh_AxleLoad4 prio=1 dataSetName=std dataClassType=initIO dataClassName=initIO unit=kg description='mec_veh_AxleLoad4': pneAux.mec_veh_AxleLoad4_0 [-]"; p121 "mec_veh_TrailerAxleLoad1 (init) export=true name=mec_veh_TrailerAxleLoad1 prio=1 dataSetName=std dataClassType=initIO dataClassName=initIO unit=kg description='mec_veh_TrailerAxleLoad1': pneAux.mec_veh_TrailerAxleLoad1_0 [-]"; p122 "mec_veh_TrailerAxleLoad2 (init) export=true name=mec_veh_TrailerAxleLoad2 prio=1 dataSetName=std dataClassType=initIO dataClassName=initIO unit=kg description='mec_veh_TrailerAxleLoad2': pneAux.mec_veh_TrailerAxleLoad2_0 [-]"; p123 "mec_veh_TrailerAxleLoad3 (init) export=true name=mec_veh_TrailerAxleLoad3 prio=1 dataSetName=std dataClassType=initIO dataClassName=initIO unit=kg description='mec_veh_TrailerAxleLoad3': pneAux.mec_veh_TrailerAxleLoad3_0 [-]"; p124 "mec_veh_transVel export=true name=mec_veh_transVel prio=1 dataSetName=std dataClassType=initIO dataClassName=initIO unit='-' description='mec_veh_transVel': pneAux.mec_veh_transVel_0 [-]"; p125 "MTBVehicleParameter (0-disabled, 1 enabled) export=true name=MTBVehicleParameter  prio=1 dataSetName=pneAux_dummy dataClassType=main dataClassName=main unit='-' description='MTBVehicleParameter (0-disabled, 1 enabled) ': pneAux.MTBVehicleParameter [-]"; p126 "PB_Sw_Stat_SATP, Parking brake button: 0,1,2,3 / Not Pressed, Pressed, ERR, SNA) export=true name=PB_Sw_Stat_SATP prio=1 dataSetName=std dataClassType=initIO dataClassName=initIO unit='-' description='Parking brake button: 0,1,2,3 / Not Pressed, Pressed, ERR, SNA)': pneAux.PB_Sw_Stat_SATP_0 [-]"; p127 "PB_Trlr_Ctrl_Stat (init) (Parking Brake Trailer Control Current state,0:notAvailable,1:Available,2:error,3:SNA) export=true name=PB_Trlr_Ctrl_Stat prio=1 dataSetName=std dataClassType=initIO dataClassName=initIO unit='-' description='PB_Trlr_Ctrl_Stat (Parking Brake Trailer Control Current state,0:notAvailable,1:Available,2:error,3:SNA)': pneAux.PB_Trlr_Ctrl_Stat_0 [-]"; p128 "PBL_Fct_Stat (init) (Parking Brake Lever Function Current state,0:parkingBrake,1:TrailerBrake,2:error,3:SNA) export=true name=PBL_Fct_Stat prio=1 dataSetName=std dataClassType=initIO dataClassName=initIO unit='-' description='PBL_Fct_Stat (Parking Brake Lever Function Current state,0:parkingBrake,1:TrailerBrake,2:error,3:SNA)': pneAux.PBL_Fct_Stat_0 [-]"; p129 "PBL_LvrPosn_Cval (init) Parking Brake Lever Lever Position Current value export=true name=PBL_LvrPosn_Cval prio=1 dataSetName=std dataClassType=initIO dataClassName=initIO unit=% description='PBL_LvrPosn_Cval Parking Brake Lever Lever Position Current value': pneAux.PBL_LvrPosn_Cval_0 [-]"; p130 "PkB_TrlrAirPress_Stat_ICUC (init) export=true name=PkB_TrlrAirPress_Stat_ICUC prio=1 dataSetName=std dataClassType=initIO dataClassName=initIO unit=kPa description='PkB_TrlrAirPress_Stat_ICUC': pneAux.PkB_TrlrAirPress_Stat_ICUC_0 [-]"; p131 "PkBrk_Engg_Stat (init) (Park(ing) Brake(ing) Engaged Current state,0:notActive,1:active,2:error,3:SNA) export=true name=PkBrk_Engg_Stat prio=1 dataSetName=std dataClassType=initIO dataClassName=initIO unit='-' description='PkBrk_Engg_Stat (Park(ing) Brake(ing) Engaged Current state,0:notActive,1:active,2:error,3:SNA)': pneAux.PkBrk_Engg_Stat_0 [-]"; p132 "PkBrk_Stat_EAPU (init) (Parking Brake Current state,0:Disengaged,1:engaged,2:error,3:SNA) export=true name=PkBrk_Stat_EAPU prio=1 dataSetName=std dataClassType=initIO dataClassName=initIO unit='-' description='PkBrk_Stat_EAPU (Parking Brake Current state,0:Disengaged,1:engaged,2:error,3:SNA)': pneAux.PkBrk_Stat_EAPU_0 [-]"; p133 "PkBrk_Stat_SCH (init) (Parking Brake Current state SAM_CHAS,0:Disengaged,1:engaged,2:error,3:SNA) export=true name=PkBrk_Stat_SCH prio=1 dataSetName=std dataClassType=initIO dataClassName=initIO unit='-' description='PkBrk_Stat_SCH (Parking Brake Current state SAM_CHAS,0:Disengaged,1:engaged,2:error,3:SNA)': pneAux.PkBrk_Stat_SCH_0 [-]"; p134 "PkBrkPress_Cval (init) (Parking Brake Pressure Current value) export=true name=PkBrkPress_Cval prio=1 dataSetName=std dataClassType=initIO dataClassName=initIO unit=kPa description='PkBrkPress_Cval (Parking Brake Pressure Current value)': pneAux.PkBrkPress_Cval_0 [-]"; p135 "pne_brk_Axle1_torque_sns export=true name=pne_brk_Axle1_torque_sns prio=1 dataSetName=std dataClassType=initIO dataClassName=initIO unit='-' description='pne_brk_Axle1_torque_sns': pneAux.pne_brk_Axle1_torque_sns_0 [-]"; p136 "pne_brk_Axle2_torque_sns export=true name=pne_brk_Axle2_torque_sns prio=1 dataSetName=std dataClassType=initIO dataClassName=initIO unit='-' description='pne_brk_Axle2_torque_sns': pneAux.pne_brk_Axle2_torque_sns_0 [-]"; p137 "pne_brk_Axle3_torque_sns export=true name=pne_brk_Axle3_torque_sns prio=1 dataSetName=std dataClassType=initIO dataClassName=initIO unit='-' description='pne_brk_Axle3_torque_sns': pneAux.pne_brk_Axle3_torque_sns_0 [-]"; p138 "pne_brk_Axle4_torque_sns export=true name=pne_brk_Axle4_torque_sns prio=1 dataSetName=std dataClassType=initIO dataClassName=initIO unit='-' description='pne_brk_Axle4_torque_sns': pneAux.pne_brk_Axle4_torque_sns_0 [-]"; p139 "pne_brk_BrkWearAALt export=true name=pne_brk_BrkWearAALt prio=1 dataSetName=std dataClassType=initIO dataClassName=initIO unit='%' description='pne_brk_BrkWearAALt': pneAux.pne_brk_BrkWearAALt_0 [-]"; p140 "pne_brk_BrkWearAARt export=true name=pne_brk_BrkWearAARt prio=1 dataSetName=std dataClassType=initIO dataClassName=initIO unit='%' description='pne_brk_BrkWearAARt': pneAux.pne_brk_BrkWearAARt_0 [-]"; p141 "pne_brk_BrkWearFA1Lt export=true name=pne_brk_BrkWearFA1Lt prio=1 dataSetName=std dataClassType=initIO dataClassName=initIO unit='%' description='pne_brk_BrkWearFA1Lt': pneAux.pne_brk_BrkWearFA1Lt_0 [-]"; p142 "pne_brk_BrkWearFA1Rt export=true name=pne_brk_BrkWearFA1Rt prio=1 dataSetName=std dataClassType=initIO dataClassName=initIO unit='%' description='pne_brk_BrkWearFA1Rt': pneAux.pne_brk_BrkWearFA1Rt_0 [-]"; p143 "pne_brk_BrkWearFA2Lt export=true name=pne_brk_BrkWearFA2Lt prio=1 dataSetName=std dataClassType=initIO dataClassName=initIO unit='%' description='pne_brk_BrkWearFA2Lt': pneAux.pne_brk_BrkWearFA2Lt_0 [-]"; p144 "pne_brk_BrkWearFA2Rt export=true name=pne_brk_BrkWearFA2Rt prio=1 dataSetName=std dataClassType=initIO dataClassName=initIO unit='%' description='pne_brk_BrkWearFA2Rt': pneAux.pne_brk_BrkWearFA2Rt_0 [-]"; p145 "pne_brk_BrkWearRA1Lt export=true name=pne_brk_BrkWearRA1Lt prio=1 dataSetName=std dataClassType=initIO dataClassName=initIO unit='%' description='pne_brk_BrkWearRA1Lt': pneAux.pne_brk_BrkWearRA1Lt_0 [-]"; p146 "pne_brk_BrkWearRA1Rt export=true name=pne_brk_BrkWearRA1Rt prio=1 dataSetName=std dataClassType=initIO dataClassName=initIO unit='%' description='pne_brk_BrkWearRA1Rt': pneAux.pne_brk_BrkWearRA1Rt_0 [-]"; p147 "pne_brk_BrkWearRA2Lt export=true name=pne_brk_BrkWearRA2Lt prio=1 dataSetName=std dataClassType=initIO dataClassName=initIO unit='%' description='pne_brk_BrkWearRA2Lt': pneAux.pne_brk_BrkWearRA2Lt_0 [-]"; p148 "pne_brk_BrkWearRA2Rt export=true name=pne_brk_BrkWearRA2Rt prio=1 dataSetName=std dataClassType=initIO dataClassName=initIO unit='%' description='pne_brk_BrkWearRA2Rt': pneAux.pne_brk_BrkWearRA2Rt_0 [-]"; p149 "Compressor ON (1 - ON, 0 - OFF) (init) export=true name=pne_brk_CompON prio=1 dataSetName=std dataClassType=initIO dataClassName=initIO unit='-' description='Compressor ON (1 - ON, 0 - OFF) (init)': pneAux.pne_brk_CompON_0 [-]"; p150 "Pressure (relative) Spring Brake [bar] (init) export=true name=pne_brk_pRelPkBrk prio=1 dataSetName=std dataClassType=initIO dataClassName=initIO unit=bar description='Pressure (relative) Spring Brake [bar] (init) ': pneAux.pne_brk_pRelPkBrk_0 [-]"; p151 "pne_brk_reg_active (init) export=true name=pne_brk_reg_active prio=1 dataSetName=std dataClassType=initIO dataClassName=initIO unit='-' description='Regeneraaton active': pneAux.pne_brk_reg_active_0 [-]"; p152 "wheel speed trailer axle1 left wheel (init) export=true name=pne_brk_rotVel_t1l prio=1 dataSetName=std dataClassType=initIO dataClassName=initIO unit='-' description='wheel speed trailer axle1 left wheel': pneAux.pne_brk_rotVel_t1l_0 [-]"; p153 "wheel speed trailer axle1 right wheel (init) export=true name=pne_brk_rotVel_t1r prio=1 dataSetName=std dataClassType=initIO dataClassName=initIO unit='-' description='wheel speed trailer axle3 right wheel': pneAux.pne_brk_rotVel_t1r_0 [-]"; p154 "wheel speed trailer axle2 left wheel (init) export=true name=pne_brk_rotVel_t2l prio=1 dataSetName=std dataClassType=initIO dataClassName=initIO unit='-' description='wheel speed trailer axle2 left wheel': pneAux.pne_brk_rotVel_t2l_0 [-]"; p155 "wheel speed trailer axle2 right wheel (init) export=true name=pne_brk_rotVel_t2r prio=1 dataSetName=std dataClassType=initIO dataClassName=initIO unit='-' description='wheel speed trailer axle3 right wheel': pneAux.pne_brk_rotVel_t2r_0 [-]"; p156 "wheel speed trailer axle3 left wheel (init) export=true name=pne_brk_rotVel_t3l prio=1 dataSetName=std dataClassType=initIO dataClassName=initIO unit='-' description='wheel speed trailer axle3 left wheel': pneAux.pne_brk_rotVel_t3l_0 [-]"; p157 "wheel speed trailer axle3 right wheel (init) export=true name=pne_brk_rotVel_t3r prio=1 dataSetName=std dataClassType=initIO dataClassName=initIO unit='-' description='wheel speed trailer axle3 right wheel': pneAux.pne_brk_rotVel_t3r_0 [-]"; p158 "pne_brk_Trailer_RV_Front_pAct (init) export=true name=pne_brk_Trailer_RV_Front_pAct prio=1 dataSetName=std dataClassType=initIO dataClassName=initIO unit='-' description='pne_brk_Trailer_RV_Front_pAct'': pneAux.pne_brk_Trailer_RV_Front_pAct_0 [-]"; p159 "pne_brk_Trailer_RV_Rear_pAct (init) export=true name=pne_brk_Trailer_RV_Rear_pAct prio=1 dataSetName=std dataClassType=initIO dataClassName=initIO unit='-' description='pne_brk_Trailer_RV_Rear_pAct'': pneAux.pne_brk_Trailer_RV_Rear_pAct_0 [-]"; p160 "pne_brk_TrailerAxle1_BrakingForce_at8p5bar (init) export=true name=pne_brk_TrailerAxle1_BrakingForce_at8p5bar prio=1 dataSetName=std dataClassType=initIO dataClassName=initIO unit=N description='pne_brk_TrailerAxle1_BrakingForce_at8p5bar': pneAux.pne_brk_TrailerAxle1_BrakingForce_at8p5bar_0 [-]"; p161 "pne_brk_TrailerAxle1_torque_sns export=true name=pne_brk_TrailerAxle1_torque_sns prio=1 dataSetName=std dataClassType=initIO dataClassName=initIO unit='-' description='pne_brk_TrailerAxle1_torque_sns': pneAux.pne_brk_TrailerAxle1_torque_sns_0 [-]"; p162 "pne_brk_TrailerAxle2_BrakingForce_at8p5bar (init) export=true name=pne_brk_TrailerAxle2_BrakingForce_at8p5bar prio=1 dataSetName=std dataClassType=initIO dataClassName=initIO unit=N description='pne_brk_TrailerAxle2_BrakingForce_at8p5bar': pneAux.pne_brk_TrailerAxle2_BrakingForce_at8p5bar_0 [-]"; p163 "pne_brk_TrailerAxle2_torque_sns export=true name=pne_brk_TrailerAxle2_torque_sns prio=1 dataSetName=std dataClassType=initIO dataClassName=initIO unit='-' description='pne_brk_TrailerAxle2_torque_sns': pneAux.pne_brk_TrailerAxle2_torque_sns_0 [-]"; p164 "pne_brk_TrailerAxle3_BrakingForce_at8p5bar (init) export=true name=pne_brk_TrailerAxle3_BrakingForce_at8p5bar prio=1 dataSetName=std dataClassType=initIO dataClassName=initIO unit=N description='pne_brk_TrailerAxle3_BrakingForce_at8p5bar': pneAux.pne_brk_TrailerAxle3_BrakingForce_at8p5bar_0 [-]"; p165 "pne_brk_TrailerAxle3_torque_sns export=true name=pne_brk_TrailerAxle3_torque_sns prio=1 dataSetName=std dataClassType=initIO dataClassName=initIO unit='-' description='pne_brk_TrailerAxle3_torque_sns': pneAux.pne_brk_TrailerAxle3_torque_sns_0 [-]"; p166 "Relative Pressure Tank1 [bar] (init) export=true name=pne_brk_V1_pRel prio=1 dataSetName=std dataClassType=initIO dataClassName=initIO unit=bar description='Relative Pressure Tank1 [bar] (init) ': pneAux.pne_brk_V1_pRel_0 [-]"; p167 "Relative Pressure Tank2 [bar] (init) export=true name=pne_brk_V2_pRel prio=1 dataSetName=std dataClassType=initIO dataClassName=initIO unit=bar description='Relative Pressure Tank2 [bar] (init) ': pneAux.pne_brk_V2_pRel_0 [-]"; p168 "Relative Pressure Tank4 [bar] (init) export=true name=pne_brk_V4_pRel prio=1 dataSetName=std dataClassType=initIO dataClassName=initIO unit=bar description='Relative Pressure Tank4 [bar] (init) ': pneAux.pne_brk_V4_pRel_0 [-]"; p169 "pne_brk_V7_pRel (init) export=true name=pne_brk_V7_pRel prio=1 dataSetName=std dataClassType=initIO dataClassName=initIO unit='bar' description='Relative Pressure Tank7 [bar]': pneAux.pne_brk_V7_pRel_0 [-]"; p170 "Relative Pressure Tank Trailer [bar] (init) export=true name=pne_brk_VTrailer_pRel prio=1 dataSetName=std dataClassType=initIO dataClassName=initIO unit=bar description='Relative Pressure Tank Trailer [bar] (init) ': pneAux.pne_brk_VTrailer_pRel_0 [-]"; p171 "pne_brk_WetLvl_Cntr (init) export=true name=pne_brk_WetLvl_Cntr prio=1 dataSetName=std dataClassType=initIO dataClassName=initIO unit='Nl' description='Calculated Wettnesslevel of the cartridge / Nl': pneAux.pne_brk_WetLvl_Cntr_0 [-]"; p172 "pne_MTBmodusSwAllowed (init) export=true name=pne_MTBmodusSwAllowed prio=1 dataSetName=std dataClassType=initIO dataClassName=initIO unit='-' description='pne_MTBmodusSwAllowed': pneAux.pne_MTBmodusSwAllowed_0 [-]"; p173 "pne_susp_A1_Le_Posn [mm] (init) export=true name=pne_susp_A1_Le_Posn prio=1 dataSetName=std dataClassType=initIO dataClassName=initIO unit='-' description='pne_susp_A1_Le_Posn [mm]': pneAux.pne_susp_A1_Le_Posn_0 [-]"; p174 "pne_susp_A1_Ri_Posn [mm] (init) export=true name=pne_susp_A1_Ri_Posn prio=1 dataSetName=std dataClassType=initIO dataClassName=initIO unit='-' description='pne_susp_A1_Ri_Posn [mm]': pneAux.pne_susp_A1_Ri_Posn_0 [-]"; p175 "pne_susp_A2_Le_Posn [mm] (init) export=true name=pne_susp_A2_Le_Posn prio=1 dataSetName=std dataClassType=initIO dataClassName=initIO unit='-' description='pne_susp_A2_Le_Posn [mm]': pneAux.pne_susp_A2_Le_Posn_0 [-]"; p176 "pne_susp_A2_Ri_Posn [mm] (init) export=true name=pne_susp_A2_Ri_Posn prio=1 dataSetName=std dataClassType=initIO dataClassName=initIO unit='-' description='pne_susp_A2_Ri_Posn [mm]': pneAux.pne_susp_A2_Ri_Posn_0 [-]"; p177 "pne_susp_A3_Le_Posn [mm] (init) export=true name=pne_susp_A3_Le_Posn prio=1 dataSetName=std dataClassType=initIO dataClassName=initIO unit='-' description='pne_susp_A3_Le_Posn [mm]': pneAux.pne_susp_A3_Le_Posn_0 [-]"; p178 "pne_susp_A3_Ri_Posn [mm] (init) export=true name=pne_susp_A3_Ri_Posn prio=1 dataSetName=std dataClassType=initIO dataClassName=initIO unit='-' description='pne_susp_A3_Ri_Posn [mm]': pneAux.pne_susp_A3_Ri_Posn_0 [-]"; p179 "pneAux_A1_Le_Rq (init) export=true name=pneAux_A1_Le_Rq prio=1 dataSetName=std dataClassType=initIO dataClassName=initIO unit='-' description='pneAux_A1_Le_Rq': pneAux.pneAux_A1_Le_Rq_0 [-]"; p180 "pneAux_A1_LoLi_Rq (init) export=true name=pneAux_A1_LoLi_Rq prio=1 dataSetName=std dataClassType=initIO dataClassName=initIO unit='-' description='pneAux_A1_LoLi_Rq': pneAux.pneAux_A1_LoLi_Rq_0 [-]"; p181 "pneAux_A1_Ri_Rq (init) export=true name=pneAux_A1_Ri_Rq prio=1 dataSetName=std dataClassType=initIO dataClassName=initIO unit='-' description='pneAux_A1_Ri_Rq': pneAux.pneAux_A1_Ri_Rq_0 [-]"; p182 "pneAux_A2_Le_Rq (init) export=true name=pneAux_A2_Le_Rq prio=1 dataSetName=std dataClassType=initIO dataClassName=initIO unit='-' description='pneAux_A2_Le_Rq': pneAux.pneAux_A2_Le_Rq_0 [-]"; p183 "pneAux_A2_LoLi_Rq (init) export=true name=pneAux_A2_LoLi_Rq prio=1 dataSetName=std dataClassType=initIO dataClassName=initIO unit='-' description='pneAux_A2_LoLi_Rq': pneAux.pneAux_A2_LoLi_Rq_0 [-]"; p184 "pneAux_A2_Ri_Rq (init) export=true name=pneAux_A2_Ri_Rq prio=1 dataSetName=std dataClassType=initIO dataClassName=initIO unit='-' description='pneAux_A2_Ri_Rq': pneAux.pneAux_A2_Ri_Rq_0 [-]"; p185 "pneAux_A3_Le_Rq (init) export=true name=pneAux_A3_Le_Rq prio=1 dataSetName=std dataClassType=initIO dataClassName=initIO unit='-' description='pneAux_A3_Le_Rq': pneAux.pneAux_A3_Le_Rq_0 [-]"; p186 "pneAux_A3_LoLi_Rq (init) export=true name=pneAux_A3_LoLi_Rq prio=1 dataSetName=std dataClassType=initIO dataClassName=initIO unit='-' description='pneAux_A3_LoLi_Rq': pneAux.pneAux_A3_LoLi_Rq_0 [-]"; p187 "pneAux_A3_Ri_Rq (init) export=true name=pneAux_A3_Ri_Rq prio=1 dataSetName=std dataClassType=initIO dataClassName=initIO unit='-' description='pneAux_A3_Ri_Rq': pneAux.pneAux_A3_Ri_Rq_0 [-]"; p188 "pneAux_Axle1_load (init) export=true name=pneAux_Axle1_load prio=1 dataSetName=std dataClassType=initIO dataClassName=initIO unit=kg description='pneAux_Axle1_load': pneAux.pneAux_Axle1_load_0 [-]"; p189 "pneAux_Axle2_load (init) export=true name=pneAux_Axle2_load prio=1 dataSetName=std dataClassType=initIO dataClassName=initIO unit=kg description='pneAux_Axle2_load': pneAux.pneAux_Axle2_load_0 [-]"; p190 "pneAux_Axle3_load (init) export=true name=pneAux_Axle3_load prio=1 dataSetName=std dataClassType=initIO dataClassName=initIO unit=kg description='pneAux_Axle3_load': pneAux.pneAux_Axle3_load_0 [-]"; p191 "pneAux_Axle4_load (init) export=true name=pneAux_Axle4_load prio=1 dataSetName=std dataClassType=initIO dataClassName=initIO unit=kg description='pneAux_Axle4_load': pneAux.pneAux_Axle4_load_0 [-]"; p192 "pneAux_Drs_Rq (init) export=true name=pneAux_Drs_Rq prio=1 dataSetName=std dataClassType=initIO dataClassName=initIO unit='-' description='pneAux_Drs_Rq': pneAux.pneAux_Drs_Rq_0 [-]"; p193 "pneAux_EAPU_overrun (init) export=true name=pneAux_EAPU_overrun prio=1 dataSetName=std dataClassType=initIO dataClassName=initIO unit='-' description='pneAux_EAPU_overrun (init)': pneAux.pneAux_EAPU_overrun_0 [-]"; p194 "pneAux_mass_Tractor (init) export=true name=pneAux_mass_Tractor prio=1 dataSetName=std dataClassType=initIO dataClassName=initIO unit=kg description='pneAux_mass_Tractor': pneAux.pneAux_mass_Tractor_0 [-]"; p195 "pneAux_mass_Trailer (init) export=true name=pneAux_mass_Trailer prio=1 dataSetName=std dataClassType=initIO dataClassName=initIO unit=kg description='pneAux_mass_Trailer': pneAux.pneAux_mass_Trailer_0 [-]"; p196 "pneAux_pSoll_TCV_p43 (init) export=true name=pneAux_pSoll_TCV_p43 prio=1 dataSetName=std dataClassType=initIO dataClassName=initIO unit='-' description='pneAux_pSoll_TCV_p43 (init)': pneAux.pneAux_pSoll_TCV_p43_0 [-]"; p197 "pneAux_pSollPkBrk (init) export=true name=pneAux_pSollPkBrk prio=1 dataSetName=std dataClassType=initIO dataClassName=initIO unit='-' description='pneAux_pSollPkBrk (init)': pneAux.pneAux_pSollPkBrk_0 [-]"; p198 "pneAux_SumBrakingForces_Tractor (init) export=true name=pneAux_SumBrakingForces_Tractor prio=1 dataSetName=std dataClassType=initIO dataClassName=initIO unit=N description='pneAux_SumBrakingForces_Tractor': pneAux.pneAux_SumBrakingForces_Tractor_0 [-]"; p199 "pneAux_SumBrakingForces_Trailer (init) export=true name=pneAux_SumBrakingForces_Trailer prio=1 dataSetName=std dataClassType=initIO dataClassName=initIO unit=N description='pneAux_SumBrakingForces_Trailer': pneAux.pneAux_SumBrakingForces_Trailer_0 [-]"; p200 "pneAux_TCV_pDmd_Front_Left (init) export=true name=pneAux_TCV_pDmd_Front_Left prio=1 dataSetName=std dataClassType=initIO dataClassName=initIO unit='-' description='pneAux_TCV_pDmd_Front_Right': pneAux.pneAux_TCV_pDmd_Front_Left_0 [-]"; p201 "pneAux_TCV_pDmd_Front_Right (init) export=true name=pneAux_TCV_pDmd_Front_Right prio=1 dataSetName=std dataClassType=initIO dataClassName=initIO unit='-' description='pneAux_TCV_pDmd_Front_Right': pneAux.pneAux_TCV_pDmd_Front_Right_0 [-]"; p202 "pneAux_TCV_pDmd_Rear_Left (init) export=true name=pneAux_TCV_pDmd_Rear_Left prio=1 dataSetName=std dataClassType=initIO dataClassName=initIO unit='-' description='pneAux_TCV_pDmd_Front_Right': pneAux.pneAux_TCV_pDmd_Rear_Left_0 [-]"; p203 "pneAux_TCV_pDmd_Rear_Right (init) export=true name=pneAux_TCV_pDmd_Rear_Right prio=1 dataSetName=std dataClassType=initIO dataClassName=initIO unit='-' description='pneAux_TCV_pDmd_Front_Right': pneAux.pneAux_TCV_pDmd_Rear_Right_0 [-]"; p204 "pneAux_trailerAxle1_left_stABSInValve export=true name=pneAux_trailerAxle1_left_stABSInValve prio=1 dataSetName=std dataClassType=initIO dataClassName=initIO unit='-' description='pneAux_trailerAxle1_left_stABSInValve': pneAux.pneAux_trailerAxle1_left_stABSInValve_0 [-]"; p205 "pneAux_trailerAxle1_left_stABSOutValve export=true name=pneAux_trailerAxle1_left_stABSOutValve prio=1 dataSetName=std dataClassType=initIO dataClassName=initIO unit='-' description='pneAux_trailerAxle1_left_stABSOutValve': pneAux.pneAux_trailerAxle1_left_stABSOutValve_0 [-]"; p206 "pneAux_trailerAxle1_load (init) export=true name=pneAux_trailerAxle1_load prio=1 dataSetName=std dataClassType=initIO dataClassName=initIO unit=kg description='pneAux_trailerAxle1_load': pneAux.pneAux_trailerAxle1_load_0 [-]"; p207 "pneAux_trailerAxle1_right_stABSInValve export=true name=pneAux_trailerAxle1_right_stABSInValve prio=1 dataSetName=std dataClassType=initIO dataClassName=initIO unit='-' description='pneAux_trailerAxle1_right_stABSInValve': pneAux.pneAux_trailerAxle1_right_stABSInValve_0 [-]"; p208 "pneAux_trailerAxle1_right_stABSOutValve export=true name=pneAux_trailerAxle1_right_stABSOutValve prio=1 dataSetName=std dataClassType=initIO dataClassName=initIO unit='-' description='pneAux_trailerAxle1_right_stABSOutValve': pneAux.pneAux_trailerAxle1_right_stABSOutValve_0 [-]"; p209 "pneAux_trailerAxle2_left_stABSInValve export=true name=pneAux_trailerAxle2_left_stABSInValve prio=1 dataSetName=std dataClassType=initIO dataClassName=initIO unit='-' description='pneAux_trailerAxle2_left_stABSInValve': pneAux.pneAux_trailerAxle2_left_stABSInValve_0 [-]"; p210 "pneAux_trailerAxle2_left_stABSOutValve export=true name=pneAux_trailerAxle2_left_stABSOutValve prio=1 dataSetName=std dataClassType=initIO dataClassName=initIO unit='-' description='pneAux_trailerAxle2_left_stABSOutValve': pneAux.pneAux_trailerAxle2_left_stABSOutValve_0 [-]"; p211 "pneAux_trailerAxle2_load (init) export=true name=pneAux_trailerAxle2_load prio=1 dataSetName=std dataClassType=initIO dataClassName=initIO unit=kg description='pneAux_trailerAxle2_load': pneAux.pneAux_trailerAxle2_load_0 [-]"; p212 "pneAux_trailerAxle2_right_stABSInValve export=true name=pneAux_trailerAxle2_right_stABSInValve prio=1 dataSetName=std dataClassType=initIO dataClassName=initIO unit='-' description='pneAux_trailerAxle2_right_stABSInValve': pneAux.pneAux_trailerAxle2_right_stABSInValve_0 [-]"; p213 "pneAux_trailerAxle2_right_stABSOutValve export=true name=pneAux_trailerAxle2_right_stABSOutValve prio=1 dataSetName=std dataClassType=initIO dataClassName=initIO unit='-' description='pneAux_trailerAxle2_right_stABSOutValve': pneAux.pneAux_trailerAxle2_right_stABSOutValve_0 [-]"; p214 "pneAux_trailerAxle3_left_stABSInValve export=true name=pneAux_trailerAxle3_left_stABSInValve prio=1 dataSetName=std dataClassType=initIO dataClassName=initIO unit='-' description='pneAux_trailerAxle3_left_stABSInValve': pneAux.pneAux_trailerAxle3_left_stABSInValve_0 [-]"; p215 "pneAux_trailerAxle3_left_stABSOutValve export=true name=pneAux_trailerAxle3_left_stABSOutValve prio=1 dataSetName=std dataClassType=initIO dataClassName=initIO unit='-' description='pneAux_trailerAxle3_left_stABSOutValve': pneAux.pneAux_trailerAxle3_left_stABSOutValve_0 [-]"; p216 "pneAux_trailerAxle3_load (init) export=true name=pneAux_trailerAxle3_load prio=1 dataSetName=std dataClassType=initIO dataClassName=initIO unit=kg description='pneAux_trailerAxle3_load': pneAux.pneAux_trailerAxle3_load_0 [-]"; p217 "pneAux_trailerAxle3_right_stABSInValve export=true name=pneAux_trailerAxle3_right_stABSInValve prio=1 dataSetName=std dataClassType=initIO dataClassName=initIO unit='-' description='pneAux_trailerAxle3_right_stABSInValve': pneAux.pneAux_trailerAxle3_right_stABSInValve_0 [-]"; p218 "pneAux_trailerAxle3_right_stABSOutValve export=true name=pneAux_trailerAxle3_right_stABSOutValve prio=1 dataSetName=std dataClassType=initIO dataClassName=initIO unit='-' description='pneAux_trailerAxle3_right_stABSOutValve': pneAux.pneAux_trailerAxle3_right_stABSOutValve_0 [-]"; p219 "Compressor ON (1 - ON, 0 - OFF) (init) export=true name=PressAir_Rq prio=1 dataSetName=std dataClassType=initIO dataClassName=initIO unit='-' description='Compressor ON (1 - ON, 0 - OFF) (init)': pneAux.PressAir_Rq_0 [-]"; p220 "Compressor ON (1 - ON, 0 - OFF) (init) export=true name=PressAir_Rq_ICUC prio=1 dataSetName=std dataClassType=initIO dataClassName=initIO unit='-' description='Compressor ON (1 - ON, 0 - OFF) (init)': pneAux.PressAir_Rq_ICUC_0 [-]"; p221 "PressAir_Rq_SATP, Compressor ON [0 - ON, 1 - OFF] export=true name=PressAir_Rq_SATP prio=1 dataSetName=std dataClassType=initIO dataClassName=initIO unit='-' description='Compressor ON [0 - ON, 1 - OFF]': pneAux.PressAir_Rq_SATP_0 [-]"; p222 "Switching Pressure High to Low Comp. Speed [bar] export=true name=pSwitch_bar prio=1 dataSetName=pneAux_dummy dataClassType=main dataClassName=main unit=bar description='Switching Pressure High to Low Comp. Speed [bar]': pneAux.pSwitch_bar [-]"; p223 "Dyn. Wheel Radius Front Axle [mm] export=true name=rdynFA prio=1 dataSetName=veh_dummy dataClassType=veh dataClassName=veh unit='mm' description='Dyn. Wheel Radius Front Axle [mm]': pneAux.rdynFA [-]"; p224 "Dyn. Wheel Radius Rear Axle [mm] export=true name=rdynRA prio=1 dataSetName=veh_dummy dataClassType=veh dataClassName=veh unit='mm' description='Dyn. Wheel Radius Rear Axle [mm]': pneAux.rdynRA [-]"; p225 "Dyn. Wheel Radius Trailer Axle [mm] export=true name=rdynTA prio=1 dataSetName=veh_dummy dataClassType=veh dataClassName=veh unit='mm' description='Dyn. Wheel Radius Trailer Axle [mm]': pneAux.rdynTA [-]"; p226 "RedWarn_Rq_Trlr2, Red Warning Request Trailer,0:noFailureIndicated,1:FailureIndicated,2:WariningSignalFlashing,3:SNA export=true name=RedWarn_Rq_Trlr2 prio=1 dataSetName=std dataClassType=initIO dataClassName=initIO unit='-' description='Red Warning Request Trailer,0:noFailureIndicated,1:FailureIndicated,2:WariningSignalFlashing,3:SNA': pneAux.RedWarn_Rq_Trlr2_0 [-]"; p227 "RedWarn_Rq_Trlr3,   export=true name=RedWarn_Rq_Trlr3 prio=1 dataSetName=std dataClassType=initIO dataClassName=initIO unit='-' description=' ': pneAux.RedWarn_Rq_Trlr3_0 [-]"; p228 "RedWarn_Rq_Trlr4,   export=true name=RedWarn_Rq_Trlr4 prio=1 dataSetName=std dataClassType=initIO dataClassName=initIO unit='-' description=' ': pneAux.RedWarn_Rq_Trlr4_0 [-]"; p229 "RedWarn_Rq_Trlr5,   export=true name=RedWarn_Rq_Trlr5 prio=1 dataSetName=std dataClassType=initIO dataClassName=initIO unit='-' description=' ': pneAux.RedWarn_Rq_Trlr5_0 [-]"; p230 "RedWarn_Rq_Trlr export=true name=RedWarn_Rq_Trlr prio=1 dataSetName=std dataClassType=initIO dataClassName=initIO unit='-' description='RedWarn_Rq_Trlr': pneAux.RedWarn_Rq_Trlr_0 [-]"; p231 "Step Size ABS [s] export=true name=stepSize prio=1 dataSetName=veh_dummy dataClassType=veh dataClassName=veh unit='s' description='step size [s]': pneAux.stepSize [s]"; p232 "SuspAirPress_Stat_SATP,   export=true name=SuspAirPress_Stat_SATP prio=1 dataSetName=std dataClassType=initIO dataClassName=initIO unit='-' description=' ': pneAux.SuspAirPress_Stat_SATP_0 [-]"; p233 "TBL_LvrPosn_Cval, Lever: 0..100, 101..253,254,255 / 0..100, RES,ERR,SNA export=true name=TBL_LvrPosn_Cval prio=1 dataSetName=std dataClassType=initIO dataClassName=initIO unit='%' description='Lever: 0..100, 101..253,254,255 / 0..100, RES,ERR,SNA': pneAux.TBL_LvrPosn_Cval_0 [-]"; p234 "Minimum Compressor Power-On Time [s] export=true name=tDelay prio=1 dataSetName=pneAux_dummy dataClassType=main dataClassName=main unit='s' description='Minimum Compressor Power-On Time [s]': pneAux.tDelay [-]"; p235 "Velocity Offset L1o (km/h) export=true name=TrailerABS_L1o prio=1 dataSetName=veh_dummy dataClassType=veh dataClassName=veh unit='km/h' description='Velocity Offset L1o (km/h)': pneAux.TrailerABS_L1o [-]"; p236 "Speed Fraction for Threshold Speed 1 (0.01%) export=true name=TrailerABS_L1v prio=1 dataSetName=veh_dummy dataClassType=veh dataClassName=veh unit='' description='Speed Fraction for Threshold Speed 1 (0.01%)': pneAux.TrailerABS_L1v [-]"; p237 "Velocity Offset L2o (km/h) export=true name=TrailerABS_L2o prio=1 dataSetName=veh_dummy dataClassType=veh dataClassName=veh unit='km/h' description='Velocity Offset L2o (km/h)': pneAux.TrailerABS_L2o [-]"; p238 "Speed Fraction for Threshold Speed 2 (0.01%) export=true name=TrailerABS_L2v prio=1 dataSetName=veh_dummy dataClassType=veh dataClassName=veh unit='' description='Speed Fraction for Threshold Speed 2 (0.01%)': pneAux.TrailerABS_L2v [-]"; p239 "Decceleration Threshold in [g] export=true name=TrailerABS_MinusB prio=1 dataSetName=veh_dummy dataClassType=veh dataClassName=veh unit='' description='Decceleration Threshold in [g]': pneAux.TrailerABS_MinusB [-]"; p240 "Acceleration Threshold in [g] export=true name=TrailerABS_PlusB prio=1 dataSetName=veh_dummy dataClassType=veh dataClassName=veh unit='' description='Decceleration Threshold in [g]': pneAux.TrailerABS_PlusB [-]"; p241 "Upper Acceleration Threshold in [g] export=true name=TrailerABS_PlusOB prio=1 dataSetName=veh_dummy dataClassType=veh dataClassName=veh unit='' description='Upper Acceleration Threshold in [g]': pneAux.TrailerABS_PlusOB [-]"; p242 "Holding Time [ms] export=true name=TrailerABS_THe prio=1 dataSetName=veh_dummy dataClassType=veh dataClassName=veh unit='ms' description='Holding Time [ms]': pneAux.TrailerABS_THe [-]"; p243 "Holding Time for Pulsating Pressure Build-Up [ms] export=true name=TrailerABS_TPulHold prio=1 dataSetName=veh_dummy dataClassType=veh dataClassName=veh unit='ms' description='Holding Time for Pulsating Pressure Build-Up [ms]': pneAux.TrailerABS_TPulHold [-]"; p244 "Opening Time for Pulsating Pressure Build-Up [ms] export=true name=TrailerABS_TPulOpen prio=1 dataSetName=veh_dummy dataClassType=veh dataClassName=veh unit='ms' description='Opening Time for Pulsating Pressure Build-Up [ms]': pneAux.TrailerABS_TPulOpen [-]"; p245 "Minimum Velocity for ABS Activity [km/h] export=true name=TrailerABS_vMin_kmh prio=1 dataSetName=veh_dummy dataClassType=veh dataClassName=veh unit='km/h' description='Minimum Velocity for ABS Activity [km/h]': pneAux.TrailerABS_vMin_kmh [-]"; p246 "Trlr_Air_Sup_Sw_Stat, Trailer Air Supply Switch Status for DTNA Varian: 0,1,2,3 /  Neutral, Pulled (Apply PB), Pushed (Release PB), SNA export=true name=Trlr_Air_Sup_Sw_Stat prio=1 dataSetName=std dataClassType=initIO dataClassName=initIO unit='-' description='Trailer Air Supply Switch Status for DTNA Varian: 0,1,2,3 /  Neutral, Pulled (Apply PB), Pushed (Release PB), SNA': pneAux.Trlr_Air_Sup_Sw_Stat_0 [-]"; p247 "Trlr_Air_Supply_Press_Cval, 0..250,251..253,254,255 / 0..2000, RES,ERR,SNA export=true name=Trlr_Air_Supply_Press_Cval prio=1 dataSetName=std dataClassType=initIO dataClassName=initIO unit='kPa' description='0..250,251..253,254,255 / 0..2000, RES,ERR,SNA': pneAux.Trlr_Air_Supply_Press_Cval_0 [-]"; p248 "ABS control active: 0 passive / 1 active / 2 res / 3 SNA (init) export=true name=VehABS_Stat_Trlr prio=1 dataSetName=std dataClassType=initIO dataClassName=initIO unit='-' description='ABS control active: 0 passive / 1 active / 2 res / 3 SNA': pneAux.VehABS_Stat_Trlr_0 [-]"; p249 "Wheel based Vehicel Speed Current Value Trailer (init) export=true name=VehSpd1_Cval_Trlr prio=1 dataSetName=std dataClassType=initIO dataClassName=initIO unit='-' description='Wheel based Vehicel Speed Current Value Trailer': pneAux.VehSpd1_Cval_Trlr_0 [-]"; p250 "WetLvlCntr_Cval_SATP, Cartridge wettness level / Normliter: 0..250, 254, 255 / 0..62500 physicalisch , ERR, SNA   export=true name=WetLvlCntr_Cval_SATP prio=1 dataSetName=std dataClassType=initIO dataClassName=initIO unit='l' description='Cartridge wettness level / Normliter: 0..250, 254, 255 / 0..62500 physicalisch , ERR, SNA  ': pneAux.WetLvlCntr_Cval_SATP_0 [-]"; p251 "Axle Loads Trailer export=true name=axleLoadTrailer_kg prio=1 dataSetName=veh_dummy dataClassType=veh dataClassName=veh unit=kg description='Axle Loads Trailer': pneAux.axleLoadTrailer_kg [-]"; p252 "Axle Loads Vehicle export=true name=axleLoadVehicle_kg prio=1 dataSetName=veh_dummy dataClassType=veh dataClassName=veh unit=kg description='Axle Loads Vehicle': pneAux.axleLoadVehicle_kg [-]"; p253 "Brake Circuit Configuration [A1, A2, A3, A4] (0-Dummy, 1-Front, 2-Rear, 3-Middle(Bus)) export=true name=brkCircuit prio=1 dataSetName=veh_dummy dataClassType=veh dataClassName=veh unit='-' description='Brake Circuit Configuration [A1, A2, A3, A4] (0-Dummy, 1-Front, 2-Rear, 3-Middle(Bus))': pneAux.brkCircuit [-]"; p254 "Brake Circuit Configuration {TA1, TA2, TA3} [0-Dummy, 1-Front, 2-Rear] export=true name=brkCircuitTrailer prio=1 dataSetName=veh_dummy dataClassType=veh dataClassName=veh unit='-' description='Brake Circuit Configuration Trailer {TA1, TA2, TA3} [0-Dummy, 1-Front, 2-Rear]': pneAux.brkCircuitTrailer [-]"; p255 "Trailer Control Active / Trailer can brake {flag, x1, x2, x3, x4, x5, y1, y2, y3, y4, y5} (flag: 0 - no, 1- yes ALB lower limit, 2- yes ALB normal, 3- yes ALB upper limit , 4 - yes without ALB, 5 - with characteristics {{x1 ...x5},{y1...y5}) export=true name=flagTrailerControlActive prio=1 dataSetName=veh_dummy dataClassType=veh dataClassName=veh unit='-' description='Trailer Control Active / Trailer can brake {flag, x1, x2, x3, x4, x5, y1, y2, y3, y4, y5} (flag: 0 - no, 1- yes ALB lower limit, 2- yes ALB normal, 3- yes ALB upper limit , 4 - yes without ALB, 5 - with characteristics {{x1 ...x5},{y1...y5})': pneAux.flagTrailerControlActive [-]"; p256 "application pressure of trailer axles [TA1, TA2, TA3] [bar] export=true name=pAppCyl_Trailer prio=1 dataSetName=veh_dummy dataClassType=veh dataClassName=veh unit='bar' description='application pressure of trailer axles [TA1, TA2, TA3] [bar]': pneAux.pAppCyl_Trailer [-]"; p257 "Trailer Speed Sensor Axle Position [0-false,1-true] {A1,A2,A3} export=true name=speedSensorPosnTrailer prio=1 dataSetName=veh_dummy dataClassType=veh dataClassName=veh unit='' description='Trailer Speed Sensor Axle Position [0-false,1-true] {A1,A2,A3}': pneAux.speedSensorPosnTrailer [-]"
      mask help: Generated by SimulationX 4.0.5.60286 x64
      mask init:
      | if ~isempty(initCmd), try, evalin('base', initCmd); end, end
      mask Display: disp('pneAux_rebuild_generic_std_sf'); port_label('input', 1, 'env_Temperature'); port_label('input', 2, 'ActlEngPctTrq_Cval'); port_label('input', 3, 'aSatpAutoOpMd_Cmd_SDS'); port_label('input', 4, 'BS_PB_Fct_Rq'); port_label('input', 5, 'ch_Clutch_Stat_CPC'); port_label('input', 6, 'drv_PB_Sw_Stat_SATP'); port_label('input', 7, 'drv_Trlr_Air_Sup_Sw_Stat'); port_label('input', 8, 'EngRPM_Cval_CPC3'); port_label('input', 9, 'pne_MTBmodusSwAllowed'); port_label('input', 10, 'drv_DrS_Rq'); port_label('input', 11, 'drv_Knl_Rq'); port_label('input', 12, 'drv_PkBrk'); port_label('input', 13, 'drv_PkBrkLever_pos'); port_label('input', 14, 'hvs_AirCompressor_nEmot'); port_label('input', 15, 'hvs_InverterAirCompressor_hvCurrent'); port_label('input', 16, 'hvs_InverterAirCompressor_hvVoltage'); port_label('input', 17, 'mec_veh_AxleLoad1'); port_label('input', 18, 'mec_veh_AxleLoad2'); port_label('input', 19, 'mec_veh_AxleLoad3'); port_label('input', 20, 'mec_veh_AxleLoad4'); port_label('input', 21, 'mec_veh_TrailerAxleLoad1'); port_label('input', 22, 'mec_veh_TrailerAxleLoad2'); port_label('input', 23, 'mec_veh_TrailerAxleLoad3'); port_label('input', 24, 'mec_veh_transVel'); port_label('input', 25, 'pne_brk_Axle1_torque_sns'); port_label('input', 26, 'pne_brk_Axle2_torque_sns'); port_label('input', 27, 'pne_brk_Axle3_torque_sns'); port_label('input', 28, 'pne_brk_Axle4_torque_sns'); port_label('input', 29, 'pne_brk_BrkWearAALt'); port_label('input', 30, 'pne_brk_BrkWearAARt'); port_label('input', 31, 'pne_brk_BrkWearFA1Lt'); port_label('input', 32, 'pne_brk_BrkWearFA1Rt'); port_label('input', 33, 'pne_brk_BrkWearFA2Lt'); port_label('input', 34, 'pne_brk_BrkWearFA2Rt'); port_label('input', 35, 'pne_brk_BrkWearRA1Lt'); port_label('input', 36, 'pne_brk_BrkWearRA1Rt'); port_label('input', 37, 'pne_brk_BrkWearRA2Lt'); port_label('input', 38, 'pne_brk_BrkWearRA2Rt'); port_label('input', 39, 'pne_brk_CompON'); port_label('input', 40, 'pne_brk_pRelPkBrk'); port_label('input', 41, 'pne_brk_reg_active'); port_label('input', 42, 'pne_brk_rotVel_t1l'); port_label('input', 43, 'pne_brk_rotVel_t1r'); port_label('input', 44, 'pne_brk_rotVel_t2l'); port_label('input', 45, 'pne_brk_rotVel_t2r'); port_label('input', 46, 'pne_brk_rotVel_t3l'); port_label('input', 47, 'pne_brk_rotVel_t3r'); port_label('input', 48, 'pne_brk_Trailer_RV_Front_pAct'); port_label('input', 49, 'pne_brk_Trailer_RV_Rear_pAct'); port_label('input', 50, 'pne_brk_TrailerAxle1_BrakingForce_at8p5bar'); port_label('input', 51, 'pne_brk_TrailerAxle1_torque_sns'); port_label('input', 52, 'pne_brk_TrailerAxle2_BrakingForce_at8p5bar'); port_label('input', 53, 'pne_brk_TrailerAxle2_torque_sns'); port_label('input', 54, 'pne_brk_TrailerAxle3_BrakingForce_at8p5bar'); port_label('input', 55, 'pne_brk_TrailerAxle3_torque_sns'); port_label('input', 56, 'pne_brk_V1_pRel'); port_label('input', 57, 'pne_brk_V2_pRel'); port_label('input', 58, 'pne_brk_V4_pRel'); port_label('input', 59, 'pne_brk_V7_pRel'); port_label('input', 60, 'pne_brk_VTrailer_pRel'); port_label('input', 61, 'pne_brk_WetLvl_Cntr'); port_label('input', 62, 'pne_susp_A1_Le_Posn'); port_label('input', 63, 'pne_susp_A1_Ri_Posn'); port_label('input', 64, 'pne_susp_A2_Le_Posn'); port_label('input', 65, 'pne_susp_A2_Ri_Posn'); port_label('input', 66, 'pne_susp_A3_Le_Posn'); port_label('input', 67, 'pne_susp_A3_Ri_Posn'); port_label('output', 1, 'pneAux_A1_Le_Rq'); port_label('output', 2, 'pneAux_A1_LoLi_Rq'); port_label('output', 3, 'pneAux_A1_Ri_Rq'); port_label('output', 4, 'pneAux_A2_Le_Rq'); port_label('output', 5, 'pneAux_A2_LoLi_Rq'); port_label('output', 6, 'pneAux_A2_Ri_Rq'); port_label('output', 7, 'pneAux_A3_Le_Rq'); port_label('output', 8, 'pneAux_A3_LoLi_Rq'); port_label('output', 9, 'pneAux_A3_Ri_Rq'); port_label('output', 10, 'pneAux_Axle1_load'); port_label('output', 11, 'pneAux_Axle2_load'); port_label('output', 12, 'pneAux_Axle3_load'); port_label('output', 13, 'pneAux_Axle4_load'); port_label('output', 14, 'pneAux_Drs_Rq'); port_label('output', 15, 'pneAux_EAPU_overrun'); port_label('output', 16, 'pneAux_pSoll_TCV_p43'); port_label('output', 17, 'pneAux_pSollPkBrk'); port_label('output', 18, 'pneAux_TCV_pDmd_Front_Left'); port_label('output', 19, 'pneAux_TCV_pDmd_Front_Right'); port_label('output', 20, 'pneAux_TCV_pDmd_Rear_Left'); port_label('output', 21, 'pneAux_TCV_pDmd_Rear_Right'); port_label('output', 22, 'pneAux_trailerAxle1_left_stABSInValve'); port_label('output', 23, 'pneAux_trailerAxle1_left_stABSOutValve'); port_label('output', 24, 'pneAux_trailerAxle1_load'); port_label('output', 25, 'pneAux_trailerAxle1_right_stABSInValve'); port_label('output', 26, 'pneAux_trailerAxle1_right_stABSOutValve'); port_label('output', 27, 'pneAux_trailerAxle2_left_stABSInValve'); port_label('output', 28, 'pneAux_trailerAxle2_left_stABSOutValve'); port_label('output', 29, 'pneAux_trailerAxle2_load'); port_label('output', 30, 'pneAux_trailerAxle2_right_stABSInValve'); port_label('output', 31, 'pneAux_trailerAxle2_right_stABSOutValve'); port_label('output', 32, 'pneAux_trailerAxle3_left_stABSInValve'); port_label('output', 33, 'pneAux_trailerAxle3_left_stABSOutValve'); port_label('output', 34, 'pneAux_trailerAxle3_load'); port_label('output', 35, 'pneAux_trailerAxle3_right_stABSInValve'); port_label('output', 36, 'pneAux_trailerAxle3_right_stABSOutValve'); port_label('output', 37, 'aAirComp_Stat_SATP'); port_label('output', 38, 'aAutoMd1To2Rdy_Stat_SATP'); port_label('output', 39, 'aAutoMd1To3Rdy_Stat_SATP'); port_label('output', 40, 'aAutoMd3To1Rdy_Stat_SATP'); port_label('output', 41, 'aAutoOpMd_Stat_SATP'); port_label('output', 42, 'aBrkAirPress1_Cval_SATP'); port_label('output', 43, 'aBrkAirPress1_Stat_SATP'); port_label('output', 44, 'aBrkAirPress2_Cval_SATP'); port_label('output', 45, 'aBrkAirPress2_Stat_SATP'); port_label('output', 46, 'aImplsblMdCmdErr_Stat_SATP'); port_label('output', 47, 'AirComp_Stat_SATP'); port_label('output', 48, 'AmbWarn_Rq_Trlr'); port_label('output', 49, 'AmbWarn_Rq_Trlr2'); port_label('output', 50, 'AmbWarn_Rq_Trlr3'); port_label('output', 51, 'AmbWarn_Rq_Trlr4'); port_label('output', 52, 'AmbWarn_Rq_Trlr5'); port_label('output', 53, 'aOverVoltPrim_Stat_SATP'); port_label('output', 54, 'API2_Inv2_RqSpd_Cval'); port_label('output', 55, 'aPrkBrk_ECUAir_SOH_SATP'); port_label('output', 56, 'aPrkBrk_ECUGen_SOH_SATP'); port_label('output', 57, 'aPrkBrk_SOH_SATP'); port_label('output', 58, 'aPrkBrkFltIntrlckMdChng_SATP'); port_label('output', 59, 'aPrkBrkIntrlckMdChng_SATP'); port_label('output', 60, 'aSdsIntfPrim_SOH_SATP'); port_label('output', 61, 'aTBL_LvrPosn_Cval'); port_label('output', 62, 'aTractorParkBrake_Status_SATP'); port_label('output', 63, 'aTrctrPrkBrk_AddInf_Cvl_SATP'); port_label('output', 64, 'aTrlr_Air_Supply_Press_Cval'); port_label('output', 65, 'aTrlr_Air_Supply_Stat'); port_label('output', 66, 'aTrlrSpplyLn_AddInf_Cvl_SATP'); port_label('output', 67, 'aUnderVoltPrim_Stat_SATP'); port_label('output', 68, 'AuxAirPress_Cval_SATP'); port_label('output', 69, 'AuxAirPress_Cval_Trlr'); port_label('output', 70, 'AuxAirPress_Stat_ICUC'); port_label('output', 71, 'AuxAirPress_Stat_SATP'); port_label('output', 72, 'aVehParkBrake_Status_SATP'); port_label('output', 73, 'aVehSpdIntrlckMdChng_SATP'); port_label('output', 74, 'BrkAirPress1_Cval_SATP'); port_label('output', 75, 'BrkAirPress1_Stat_ICUC'); port_label('output', 76, 'BrkAirPress1_Stat_SATP'); port_label('output', 77, 'BrkAirPress2_Cval_SATP'); port_label('output', 78, 'BrkAirPress2_Stat_ICUC'); port_label('output', 79, 'BrkAirPress2_Stat_SATP'); port_label('output', 80, 'BrkCylAirPres_FA_LW_Cval_Trlr'); port_label('output', 81, 'BrkCylAirPres_FA_RW_Cval_Trlr'); port_label('output', 82, 'BrkCylAirPres_SA_LW_Cval_Trlr'); port_label('output', 83, 'BrkCylAirPres_SA_RW_Cval_Trlr'); port_label('output', 84, 'BrkCylAirPres_TA_LW_Cval_Trlr'); port_label('output', 85, 'BrkCylAirPres_TA_RW_Cval_Trlr'); port_label('output', 86, 'BrkElCtrl_Stat_Trlr'); port_label('output', 87, 'BrkElCtrl_Stat_Trlr2'); port_label('output', 88, 'BrkElCtrl_Stat_Trlr3'); port_label('output', 89, 'BrkElCtrl_Stat_Trlr4'); port_label('output', 90, 'BrkElCtrl_Stat_Trlr5'); port_label('output', 91, 'BrkWearAALtWhl_Cval'); port_label('output', 92, 'BrkWearAARtWhl_Cval'); port_label('output', 93, 'BrkWearFA1LtWhl_Cval'); port_label('output', 94, 'BrkWearFA1RtWhl_Cval'); port_label('output', 95, 'BrkWearFA2LtWhl_Cval'); port_label('output', 96, 'BrkWearFA2RtWhl_Cval'); port_label('output', 97, 'BrkWearRA1LtWhl_Cval'); port_label('output', 98, 'BrkWearRA1RtWhl_Cval'); port_label('output', 99, 'BrkWearRA2LtWhl_Cval'); port_label('output', 100, 'BrkWearRA2RtWhl_Cval'); port_label('output', 101, 'DispPkBrkInd01_Rq_Stat'); port_label('output', 102, 'DispPkBrkInd02_Rq_Stat'); port_label('output', 103, 'DispPkBrkInd03_Rq_Stat'); port_label('output', 104, 'DispPkBrkInd04_Rq_Stat'); port_label('output', 105, 'DispPkBrkInd05_Rq_Stat'); port_label('output', 106, 'DispPkBrkInd06_Rq_Stat'); port_label('output', 107, 'DispPkBrkInd07_Rq_Stat'); port_label('output', 108, 'DispPkBrkInd08_Rq_Stat'); port_label('output', 109, 'DispPkBrkInd09_Rq_Stat'); port_label('output', 110, 'DispPkBrkInd10_Rq_Stat'); port_label('output', 111, 'DispPkBrkInd11_Rq_Stat'); port_label('output', 112, 'DispPkBrkInd12_Rq_Stat'); port_label('output', 113, 'DispPkBrkInd13_Rq_Stat'); port_label('output', 114, 'DispPkBrkInd14_Rq_Stat'); port_label('output', 115, 'DispPkBrkInd15_Rq_Stat'); port_label('output', 116, 'DispPkBrkInd16_Rq_Stat'); port_label('output', 117, 'DispPkBrkInd17_Rq_Stat'); port_label('output', 118, 'DispPkBrkInd18_Rq_Stat'); port_label('output', 119, 'ElComp_ActDischarge_Stat'); port_label('output', 120, 'ElComp_ActlSpd_Cval'); port_label('output', 121, 'ElComp_Backup_Rq'); port_label('output', 122, 'ElComp_CurrentCons_Cval'); port_label('output', 123, 'ElComp_PwrCons_Cval'); port_label('output', 124, 'ElComp_SpdMd_Stat'); port_label('output', 125, 'ElComp_Stat'); port_label('output', 126, 'ElComp_Volt_Cval'); port_label('output', 127, 'ElLoadProp_Stat_Trlr'); port_label('output', 128, 'ElLoadProp_Stat_Trlr2'); port_label('output', 129, 'ElLoadProp_Stat_Trlr3'); port_label('output', 130, 'ElLoadProp_Stat_Trlr4'); port_label('output', 131, 'ElLoadProp_Stat_Trlr5'); port_label('output', 132, 'PB_Sw_Stat_SATP'); port_label('output', 133, 'PB_Trlr_Ctrl_Stat'); port_label('output', 134, 'PBL_Fct_Stat'); port_label('output', 135, 'PBL_LvrPosn_Cval'); port_label('output', 136, 'PkB_TrlrAirPress_Stat_ICUC'); port_label('output', 137, 'PkBrk_Engg_Stat'); port_label('output', 138, 'PkBrk_Stat_EAPU'); port_label('output', 139, 'PkBrk_Stat_SCH'); port_label('output', 140, 'PkBrkPress_Cval'); port_label('output', 141, 'PressAir_Rq'); port_label('output', 142, 'PressAir_Rq_ICUC'); port_label('output', 143, 'PressAir_Rq_SATP'); port_label('output', 144, 'RedWarn_Rq_Trlr'); port_label('output', 145, 'RedWarn_Rq_Trlr2'); port_label('output', 146, 'RedWarn_Rq_Trlr3'); port_label('output', 147, 'RedWarn_Rq_Trlr4'); port_label('output', 148, 'RedWarn_Rq_Trlr5'); port_label('output', 149, 'SuspAirPress_Stat_SATP'); port_label('output', 150, 'TBL_LvrPosn_Cval'); port_label('output', 151, 'Trlr_Air_Sup_Sw_Stat'); port_label('output', 152, 'Trlr_Air_Supply_Press_Cval'); port_label('output', 153, 'VehABS_Stat_Trlr'); port_label('output', 154, 'VehSpd1_Cval_Trlr'); port_label('output', 155, 'WetLvlCntr_Cval_SATP'); port_label('output', 156, 'pneAux_mass_Tractor'); port_label('output', 157, 'pneAux_mass_Trailer'); port_label('output', 158, 'pneAux_SumBrakingForces_Tractor'); port_label('output', 159, 'pneAux_SumBrakingForces_Trailer');
  pneAux_A1_Le_Rq : Outport
  pneAux_A1_LoLi_Rq : Outport  Port=2
  pneAux_A1_Ri_Rq : Outport  Port=3
  pneAux_A2_Le_Rq : Outport  Port=4
  pneAux_A2_LoLi_Rq : Outport  Port=5
  pneAux_A2_Ri_Rq : Outport  Port=6
  pneAux_A3_Le_Rq : Outport  Port=7
  pneAux_A3_LoLi_Rq : Outport  Port=8
  pneAux_A3_Ri_Rq : Outport  Port=9
  pneAux_Axle1_load : Outport  Port=10
  pneAux_Axle2_load : Outport  Port=11
  pneAux_Axle3_load : Outport  Port=12
  pneAux_Axle4_load : Outport  Port=13
  pneAux_Drs_Rq : Outport  Port=14
  pneAux_EAPU_overrun : Outport  Port=15
  pneAux_pSoll_TCV_p43 : Outport  Port=16
  pneAux_pSollPkBrk : Outport  Port=17
  pneAux_TCV_pDmd_Front_Left : Outport  Port=18
  pneAux_TCV_pDmd_Front_Right : Outport  Port=19
  pneAux_TCV_pDmd_Rear_Left : Outport  Port=20
  pneAux_TCV_pDmd_Rear_Right : Outport  Port=21
  pneAux_trailerAxle1_left_stABSInValve : Outport  Port=22
  pneAux_trailerAxle1_left_stABSOutValve : Outport  Port=23
  pneAux_trailerAxle1_load : Outport  Port=24
  pneAux_trailerAxle1_right_stABSInValve : Outport  Port=25
  pneAux_trailerAxle1_right_stABSOutValve : Outport  Port=26
  pneAux_trailerAxle2_left_stABSInValve : Outport  Port=27
  pneAux_trailerAxle2_left_stABSOutValve : Outport  Port=28
  pneAux_trailerAxle2_load : Outport  Port=29
  pneAux_trailerAxle2_right_stABSInValve : Outport  Port=30
  pneAux_trailerAxle2_right_stABSOutValve : Outport  Port=31
  pneAux_trailerAxle3_left_stABSInValve : Outport  Port=32
  pneAux_trailerAxle3_left_stABSOutValve : Outport  Port=33
  pneAux_trailerAxle3_load : Outport  Port=34
  pneAux_trailerAxle3_right_stABSInValve : Outport  Port=35
  pneAux_trailerAxle3_right_stABSOutValve : Outport  Port=36
  aAirComp_Stat_SATP : Outport  Port=37
  aAutoMd1To2Rdy_Stat_SATP : Outport  Port=38
  aAutoMd1To3Rdy_Stat_SATP : Outport  Port=39
  aAutoMd3To1Rdy_Stat_SATP : Outport  Port=40
  aAutoOpMd_Stat_SATP : Outport  Port=41
  aBrkAirPress1_Cval_SATP : Outport  Port=42
  aBrkAirPress1_Stat_SATP : Outport  Port=43
  aBrkAirPress2_Cval_SATP : Outport  Port=44
  aBrkAirPress2_Stat_SATP : Outport  Port=45
  aImplsblMdCmdErr_Stat_SATP : Outport  Port=46
  AirComp_Stat_SATP : Outport  Port=47
  AmbWarn_Rq_Trlr : Outport  Port=48
  AmbWarn_Rq_Trlr2 : Outport  Port=49
  AmbWarn_Rq_Trlr3 : Outport  Port=50
  AmbWarn_Rq_Trlr4 : Outport  Port=51
  AmbWarn_Rq_Trlr5 : Outport  Port=52
  aOverVoltPrim_Stat_SATP : Outport  Port=53
  API2_Inv2_RqSpd_Cval : Outport  Port=54
  aPrkBrk_ECUAir_SOH_SATP : Outport  Port=55
  aPrkBrk_ECUGen_SOH_SATP : Outport  Port=56
  aPrkBrk_SOH_SATP : Outport  Port=57
  aPrkBrkFltIntrlckMdChng_SATP : Outport  Port=58
  aPrkBrkIntrlckMdChng_SATP : Outport  Port=59
  aSdsIntfPrim_SOH_SATP : Outport  Port=60
  aTBL_LvrPosn_Cval : Outport  Port=61
  aTractorParkBrake_Status_SATP : Outport  Port=62
  aTrctrPrkBrk_AddInf_Cvl_SATP : Outport  Port=63
  aTrlr_Air_Supply_Press_Cval : Outport  Port=64
  aTrlr_Air_Supply_Stat : Outport  Port=65
  aTrlrSpplyLn_AddInf_Cvl_SATP : Outport  Port=66
  aUnderVoltPrim_Stat_SATP : Outport  Port=67
  AuxAirPress_Cval_SATP : Outport  Port=68
  AuxAirPress_Cval_Trlr : Outport  Port=69
  AuxAirPress_Stat_ICUC : Outport  Port=70
  AuxAirPress_Stat_SATP : Outport  Port=71
  aVehParkBrake_Status_SATP : Outport  Port=72
  aVehSpdIntrlckMdChng_SATP : Outport  Port=73
  BrkAirPress1_Cval_SATP : Outport  Port=74
  BrkAirPress1_Stat_ICUC : Outport  Port=75
  BrkAirPress1_Stat_SATP : Outport  Port=76
  BrkAirPress2_Cval_SATP : Outport  Port=77
  BrkAirPress2_Stat_ICUC : Outport  Port=78
  BrkAirPress2_Stat_SATP : Outport  Port=79
  BrkCylAirPres_FA_LW_Cval_Trlr : Outport  Port=80
  BrkCylAirPres_FA_RW_Cval_Trlr : Outport  Port=81
  BrkCylAirPres_SA_LW_Cval_Trlr : Outport  Port=82
  BrkCylAirPres_SA_RW_Cval_Trlr : Outport  Port=83
  BrkCylAirPres_TA_LW_Cval_Trlr : Outport  Port=84
  BrkCylAirPres_TA_RW_Cval_Trlr : Outport  Port=85
  BrkElCtrl_Stat_Trlr : Outport  Port=86
  BrkElCtrl_Stat_Trlr2 : Outport  Port=87
  BrkElCtrl_Stat_Trlr3 : Outport  Port=88
  BrkElCtrl_Stat_Trlr4 : Outport  Port=89
  BrkElCtrl_Stat_Trlr5 : Outport  Port=90
  BrkWearAALtWhl_Cval : Outport  Port=91
  BrkWearAARtWhl_Cval : Outport  Port=92
  BrkWearFA1LtWhl_Cval : Outport  Port=93
  BrkWearFA1RtWhl_Cval : Outport  Port=94
  BrkWearFA2LtWhl_Cval : Outport  Port=95
  BrkWearFA2RtWhl_Cval : Outport  Port=96
  BrkWearRA1LtWhl_Cval : Outport  Port=97
  BrkWearRA1RtWhl_Cval : Outport  Port=98
  BrkWearRA2LtWhl_Cval : Outport  Port=99
  BrkWearRA2RtWhl_Cval : Outport  Port=100
  DispPkBrkInd01_Rq_Stat : Outport  Port=101
  DispPkBrkInd02_Rq_Stat : Outport  Port=102
  DispPkBrkInd03_Rq_Stat : Outport  Port=103
  DispPkBrkInd04_Rq_Stat : Outport  Port=104
  DispPkBrkInd05_Rq_Stat : Outport  Port=105
  DispPkBrkInd06_Rq_Stat : Outport  Port=106
  DispPkBrkInd07_Rq_Stat : Outport  Port=107
  DispPkBrkInd08_Rq_Stat : Outport  Port=108
  DispPkBrkInd09_Rq_Stat : Outport  Port=109
  DispPkBrkInd10_Rq_Stat : Outport  Port=110
  DispPkBrkInd11_Rq_Stat : Outport  Port=111
  DispPkBrkInd12_Rq_Stat : Outport  Port=112
  DispPkBrkInd13_Rq_Stat : Outport  Port=113
  DispPkBrkInd14_Rq_Stat : Outport  Port=114
  DispPkBrkInd15_Rq_Stat : Outport  Port=115
  DispPkBrkInd16_Rq_Stat : Outport  Port=116
  DispPkBrkInd17_Rq_Stat : Outport  Port=117
  DispPkBrkInd18_Rq_Stat : Outport  Port=118
  ElComp_ActDischarge_Stat : Outport  Port=119
  ElComp_ActlSpd_Cval : Outport  Port=120
  ElComp_Backup_Rq : Outport  Port=121
  ElComp_CurrentCons_Cval : Outport  Port=122
  ElComp_PwrCons_Cval : Outport  Port=123
  ElComp_SpdMd_Stat : Outport  Port=124
  ElComp_Stat : Outport  Port=125
  ElComp_Volt_Cval : Outport  Port=126
  ElLoadProp_Stat_Trlr : Outport  Port=127
  ElLoadProp_Stat_Trlr2 : Outport  Port=128
  ElLoadProp_Stat_Trlr3 : Outport  Port=129
  ElLoadProp_Stat_Trlr4 : Outport  Port=130
  ElLoadProp_Stat_Trlr5 : Outport  Port=131
  PB_Sw_Stat_SATP : Outport  Port=132
  PB_Trlr_Ctrl_Stat : Outport  Port=133
  PBL_Fct_Stat : Outport  Port=134
  PBL_LvrPosn_Cval : Outport  Port=135
  PkB_TrlrAirPress_Stat_ICUC : Outport  Port=136
  PkBrk_Engg_Stat : Outport  Port=137
  PkBrk_Stat_EAPU : Outport  Port=138
  PkBrk_Stat_SCH : Outport  Port=139
  PkBrkPress_Cval : Outport  Port=140
  PressAir_Rq : Outport  Port=141
  PressAir_Rq_ICUC : Outport  Port=142
  PressAir_Rq_SATP : Outport  Port=143
  RedWarn_Rq_Trlr : Outport  Port=144
  RedWarn_Rq_Trlr2 : Outport  Port=145
  RedWarn_Rq_Trlr3 : Outport  Port=146
  RedWarn_Rq_Trlr4 : Outport  Port=147
  RedWarn_Rq_Trlr5 : Outport  Port=148
  SuspAirPress_Stat_SATP : Outport  Port=149
  TBL_LvrPosn_Cval : Outport  Port=150
  Trlr_Air_Sup_Sw_Stat : Outport  Port=151
  Trlr_Air_Supply_Press_Cval : Outport  Port=152
  VehABS_Stat_Trlr : Outport  Port=153
  VehSpd1_Cval_Trlr : Outport  Port=154
  WetLvlCntr_Cval_SATP : Outport  Port=155
  pneAux_mass_Tractor : Outport  Port=156
  pneAux_mass_Trailer : Outport  Port=157
  pneAux_SumBrakingForces_Tractor : Outport  Port=158
  pneAux_SumBrakingForces_Trailer : Outport  Port=159
  wires:
  pneAux_rebuild_generic_std_sf/159 -> pneAux_SumBrakingForces_Trailer/1  "pneAux_SumBrakingForces_Trailer"
  pneAux_rebuild_generic_std_sf/158 -> pneAux_SumBrakingForces_Tractor/1  "pneAux_SumBrakingForces_Tractor"
  pneAux_rebuild_generic_std_sf/157 -> pneAux_mass_Trailer/1  "pneAux_mass_Trailer"
  pneAux_rebuild_generic_std_sf/156 -> pneAux_mass_Tractor/1  "pneAux_mass_Tractor"
  pneAux_rebuild_generic_std_sf/155 -> WetLvlCntr_Cval_SATP/1  "WetLvlCntr_Cval_SATP"
  pneAux_rebuild_generic_std_sf/154 -> VehSpd1_Cval_Trlr/1  "VehSpd1_Cval_Trlr"
  pneAux_rebuild_generic_std_sf/153 -> VehABS_Stat_Trlr/1  "VehABS_Stat_Trlr"
  pneAux_rebuild_generic_std_sf/152 -> Trlr_Air_Supply_Press_Cval/1  "Trlr_Air_Supply_Press_Cval"
  pneAux_rebuild_generic_std_sf/151 -> Trlr_Air_Sup_Sw_Stat/1  "Trlr_Air_Sup_Sw_Stat"
  pneAux_rebuild_generic_std_sf/150 -> TBL_LvrPosn_Cval/1  "TBL_LvrPosn_Cval"
  pneAux_rebuild_generic_std_sf/149 -> SuspAirPress_Stat_SATP/1  "SuspAirPress_Stat_SATP"
  pneAux_rebuild_generic_std_sf/148 -> RedWarn_Rq_Trlr5/1  "RedWarn_Rq_Trlr5"
  pneAux_rebuild_generic_std_sf/147 -> RedWarn_Rq_Trlr4/1  "RedWarn_Rq_Trlr4"
  pneAux_rebuild_generic_std_sf/146 -> RedWarn_Rq_Trlr3/1  "RedWarn_Rq_Trlr3"
  pneAux_rebuild_generic_std_sf/145 -> RedWarn_Rq_Trlr2/1  "RedWarn_Rq_Trlr2"
  pneAux_rebuild_generic_std_sf/144 -> RedWarn_Rq_Trlr/1  "RedWarn_Rq_Trlr"
  pneAux_rebuild_generic_std_sf/143 -> PressAir_Rq_SATP/1  "PressAir_Rq_SATP"
  pneAux_rebuild_generic_std_sf/142 -> PressAir_Rq_ICUC/1  "PressAir_Rq_ICUC"
  pneAux_rebuild_generic_std_sf/141 -> PressAir_Rq/1  "PressAir_Rq"
  pneAux_rebuild_generic_std_sf/140 -> PkBrkPress_Cval/1  "PkBrkPress_Cval"
  pneAux_rebuild_generic_std_sf/139 -> PkBrk_Stat_SCH/1  "PkBrk_Stat_SCH"
  pneAux_rebuild_generic_std_sf/138 -> PkBrk_Stat_EAPU/1  "PkBrk_Stat_EAPU"
  pneAux_rebuild_generic_std_sf/137 -> PkBrk_Engg_Stat/1  "PkBrk_Engg_Stat"
  pneAux_rebuild_generic_std_sf/136 -> PkB_TrlrAirPress_Stat_ICUC/1  "PkB_TrlrAirPress_Stat_ICUC"
  pneAux_rebuild_generic_std_sf/135 -> PBL_LvrPosn_Cval/1  "PBL_LvrPosn_Cval"
  pneAux_rebuild_generic_std_sf/134 -> PBL_Fct_Stat/1  "PBL_Fct_Stat"
  pneAux_rebuild_generic_std_sf/133 -> PB_Trlr_Ctrl_Stat/1  "PB_Trlr_Ctrl_Stat"
  pneAux_rebuild_generic_std_sf/132 -> PB_Sw_Stat_SATP/1  "PB_Sw_Stat_SATP"
  pneAux_rebuild_generic_std_sf/131 -> ElLoadProp_Stat_Trlr5/1  "ElLoadProp_Stat_Trlr5"
  pneAux_rebuild_generic_std_sf/130 -> ElLoadProp_Stat_Trlr4/1  "ElLoadProp_Stat_Trlr4"
  pneAux_rebuild_generic_std_sf/129 -> ElLoadProp_Stat_Trlr3/1  "ElLoadProp_Stat_Trlr3"
  pneAux_rebuild_generic_std_sf/128 -> ElLoadProp_Stat_Trlr2/1  "ElLoadProp_Stat_Trlr2"
  pneAux_rebuild_generic_std_sf/127 -> ElLoadProp_Stat_Trlr/1  "ElLoadProp_Stat_Trlr"
  pneAux_rebuild_generic_std_sf/126 -> ElComp_Volt_Cval/1  "ElComp_Volt_Cval"
  pneAux_rebuild_generic_std_sf/125 -> ElComp_Stat/1  "ElComp_Stat"
  pneAux_rebuild_generic_std_sf/124 -> ElComp_SpdMd_Stat/1  "ElComp_SpdMd_Stat"
  pneAux_rebuild_generic_std_sf/123 -> ElComp_PwrCons_Cval/1  "ElComp_PwrCons_Cval"
  pneAux_rebuild_generic_std_sf/122 -> ElComp_CurrentCons_Cval/1  "ElComp_CurrentCons_Cval"
  pneAux_rebuild_generic_std_sf/121 -> ElComp_Backup_Rq/1  "ElComp_Backup_Rq"
  pneAux_rebuild_generic_std_sf/120 -> ElComp_ActlSpd_Cval/1  "ElComp_ActlSpd_Cval"
  pneAux_rebuild_generic_std_sf/119 -> ElComp_ActDischarge_Stat/1  "ElComp_ActDischarge_Stat"
  pneAux_rebuild_generic_std_sf/118 -> DispPkBrkInd18_Rq_Stat/1  "DispPkBrkInd18_Rq_Stat"
  pneAux_rebuild_generic_std_sf/117 -> DispPkBrkInd17_Rq_Stat/1  "DispPkBrkInd17_Rq_Stat"
  pneAux_rebuild_generic_std_sf/116 -> DispPkBrkInd16_Rq_Stat/1  "DispPkBrkInd16_Rq_Stat"
  pneAux_rebuild_generic_std_sf/115 -> DispPkBrkInd15_Rq_Stat/1  "DispPkBrkInd15_Rq_Stat"
  pneAux_rebuild_generic_std_sf/114 -> DispPkBrkInd14_Rq_Stat/1  "DispPkBrkInd14_Rq_Stat"
  pneAux_rebuild_generic_std_sf/113 -> DispPkBrkInd13_Rq_Stat/1  "DispPkBrkInd13_Rq_Stat"
  pneAux_rebuild_generic_std_sf/112 -> DispPkBrkInd12_Rq_Stat/1  "DispPkBrkInd12_Rq_Stat"
  pneAux_rebuild_generic_std_sf/111 -> DispPkBrkInd11_Rq_Stat/1  "DispPkBrkInd11_Rq_Stat"
  pneAux_rebuild_generic_std_sf/110 -> DispPkBrkInd10_Rq_Stat/1  "DispPkBrkInd10_Rq_Stat"
  pneAux_rebuild_generic_std_sf/109 -> DispPkBrkInd09_Rq_Stat/1  "DispPkBrkInd09_Rq_Stat"
  pneAux_rebuild_generic_std_sf/108 -> DispPkBrkInd08_Rq_Stat/1  "DispPkBrkInd08_Rq_Stat"
  pneAux_rebuild_generic_std_sf/107 -> DispPkBrkInd07_Rq_Stat/1  "DispPkBrkInd07_Rq_Stat"
  pneAux_rebuild_generic_std_sf/106 -> DispPkBrkInd06_Rq_Stat/1  "DispPkBrkInd06_Rq_Stat"
  pneAux_rebuild_generic_std_sf/105 -> DispPkBrkInd05_Rq_Stat/1  "DispPkBrkInd05_Rq_Stat"
  pneAux_rebuild_generic_std_sf/104 -> DispPkBrkInd04_Rq_Stat/1  "DispPkBrkInd04_Rq_Stat"
  pneAux_rebuild_generic_std_sf/103 -> DispPkBrkInd03_Rq_Stat/1  "DispPkBrkInd03_Rq_Stat"
  pneAux_rebuild_generic_std_sf/102 -> DispPkBrkInd02_Rq_Stat/1  "DispPkBrkInd02_Rq_Stat"
  pneAux_rebuild_generic_std_sf/101 -> DispPkBrkInd01_Rq_Stat/1  "DispPkBrkInd01_Rq_Stat"
  pneAux_rebuild_generic_std_sf/100 -> BrkWearRA2RtWhl_Cval/1  "BrkWearRA2RtWhl_Cval"
  pneAux_rebuild_generic_std_sf/99 -> BrkWearRA2LtWhl_Cval/1  "BrkWearRA2LtWhl_Cval"
  pneAux_rebuild_generic_std_sf/98 -> BrkWearRA1RtWhl_Cval/1  "BrkWearRA1RtWhl_Cval"
  pneAux_rebuild_generic_std_sf/97 -> BrkWearRA1LtWhl_Cval/1  "BrkWearRA1LtWhl_Cval"
  pneAux_rebuild_generic_std_sf/96 -> BrkWearFA2RtWhl_Cval/1  "BrkWearFA2RtWhl_Cval"
  pneAux_rebuild_generic_std_sf/95 -> BrkWearFA2LtWhl_Cval/1  "BrkWearFA2LtWhl_Cval"
  pneAux_rebuild_generic_std_sf/94 -> BrkWearFA1RtWhl_Cval/1  "BrkWearFA1RtWhl_Cval"
  pneAux_rebuild_generic_std_sf/93 -> BrkWearFA1LtWhl_Cval/1  "BrkWearFA1LtWhl_Cval"
  pneAux_rebuild_generic_std_sf/92 -> BrkWearAARtWhl_Cval/1  "BrkWearAARtWhl_Cval"
  pneAux_rebuild_generic_std_sf/91 -> BrkWearAALtWhl_Cval/1  "BrkWearAALtWhl_Cval"
  pneAux_rebuild_generic_std_sf/90 -> BrkElCtrl_Stat_Trlr5/1  "BrkElCtrl_Stat_Trlr5"
  pneAux_rebuild_generic_std_sf/89 -> BrkElCtrl_Stat_Trlr4/1  "BrkElCtrl_Stat_Trlr4"
  pneAux_rebuild_generic_std_sf/88 -> BrkElCtrl_Stat_Trlr3/1  "BrkElCtrl_Stat_Trlr3"
  pneAux_rebuild_generic_std_sf/87 -> BrkElCtrl_Stat_Trlr2/1  "BrkElCtrl_Stat_Trlr2"
  pneAux_rebuild_generic_std_sf/86 -> BrkElCtrl_Stat_Trlr/1  "BrkElCtrl_Stat_Trlr"
  pneAux_rebuild_generic_std_sf/85 -> BrkCylAirPres_TA_RW_Cval_Trlr/1  "BrkCylAirPres_TA_RW_Cval_Trlr"
  pneAux_rebuild_generic_std_sf/84 -> BrkCylAirPres_TA_LW_Cval_Trlr/1  "BrkCylAirPres_TA_LW_Cval_Trlr"
  pneAux_rebuild_generic_std_sf/83 -> BrkCylAirPres_SA_RW_Cval_Trlr/1  "BrkCylAirPres_SA_RW_Cval_Trlr"
  pneAux_rebuild_generic_std_sf/82 -> BrkCylAirPres_SA_LW_Cval_Trlr/1  "BrkCylAirPres_SA_LW_Cval_Trlr"
  pneAux_rebuild_generic_std_sf/81 -> BrkCylAirPres_FA_RW_Cval_Trlr/1  "BrkCylAirPres_FA_RW_Cval_Trlr"
  pneAux_rebuild_generic_std_sf/80 -> BrkCylAirPres_FA_LW_Cval_Trlr/1  "BrkCylAirPres_FA_LW_Cval_Trlr"
  pneAux_rebuild_generic_std_sf/79 -> BrkAirPress2_Stat_SATP/1  "BrkAirPress2_Stat_SATP"
  pneAux_rebuild_generic_std_sf/78 -> BrkAirPress2_Stat_ICUC/1  "BrkAirPress2_Stat_ICUC"
  pneAux_rebuild_generic_std_sf/77 -> BrkAirPress2_Cval_SATP/1  "BrkAirPress2_Cval_SATP"
  pneAux_rebuild_generic_std_sf/76 -> BrkAirPress1_Stat_SATP/1  "BrkAirPress1_Stat_SATP"
  pneAux_rebuild_generic_std_sf/75 -> BrkAirPress1_Stat_ICUC/1  "BrkAirPress1_Stat_ICUC"
  pneAux_rebuild_generic_std_sf/74 -> BrkAirPress1_Cval_SATP/1  "BrkAirPress1_Cval_SATP"
  pneAux_rebuild_generic_std_sf/73 -> aVehSpdIntrlckMdChng_SATP/1  "aVehSpdIntrlckMdChng_SATP"
  pneAux_rebuild_generic_std_sf/72 -> aVehParkBrake_Status_SATP/1  "aVehParkBrake_Status_SATP"
  pneAux_rebuild_generic_std_sf/71 -> AuxAirPress_Stat_SATP/1  "AuxAirPress_Stat_SATP"
  pneAux_rebuild_generic_std_sf/70 -> AuxAirPress_Stat_ICUC/1  "AuxAirPress_Stat_ICUC"
  pneAux_rebuild_generic_std_sf/69 -> AuxAirPress_Cval_Trlr/1  "AuxAirPress_Cval_Trlr"
  pneAux_rebuild_generic_std_sf/68 -> AuxAirPress_Cval_SATP/1  "AuxAirPress_Cval_SATP"
  pneAux_rebuild_generic_std_sf/67 -> aUnderVoltPrim_Stat_SATP/1  "aUnderVoltPrim_Stat_SATP"
  pneAux_rebuild_generic_std_sf/66 -> aTrlrSpplyLn_AddInf_Cvl_SATP/1  "aTrlrSpplyLn_AddInf_Cvl_SATP"
  pneAux_rebuild_generic_std_sf/65 -> aTrlr_Air_Supply_Stat/1  "aTrlr_Air_Supply_Stat"
  pneAux_rebuild_generic_std_sf/64 -> aTrlr_Air_Supply_Press_Cval/1  "aTrlr_Air_Supply_Press_Cval"
  pneAux_rebuild_generic_std_sf/63 -> aTrctrPrkBrk_AddInf_Cvl_SATP/1  "aTrctrPrkBrk_AddInf_Cvl_SATP"
  pneAux_rebuild_generic_std_sf/62 -> aTractorParkBrake_Status_SATP/1  "aTractorParkBrake_Status_SATP"
  pneAux_rebuild_generic_std_sf/61 -> aTBL_LvrPosn_Cval/1  "aTBL_LvrPosn_Cval"
  pneAux_rebuild_generic_std_sf/60 -> aSdsIntfPrim_SOH_SATP/1  "aSdsIntfPrim_SOH_SATP"
  pneAux_rebuild_generic_std_sf/59 -> aPrkBrkIntrlckMdChng_SATP/1  "aPrkBrkIntrlckMdChng_SATP"
  pneAux_rebuild_generic_std_sf/58 -> aPrkBrkFltIntrlckMdChng_SATP/1  "aPrkBrkFltIntrlckMdChng_SATP"
  pneAux_rebuild_generic_std_sf/57 -> aPrkBrk_SOH_SATP/1  "aPrkBrk_SOH_SATP"
  pneAux_rebuild_generic_std_sf/56 -> aPrkBrk_ECUGen_SOH_SATP/1  "aPrkBrk_ECUGen_SOH_SATP"
  pneAux_rebuild_generic_std_sf/55 -> aPrkBrk_ECUAir_SOH_SATP/1  "aPrkBrk_ECUAir_SOH_SATP"
  pneAux_rebuild_generic_std_sf/54 -> API2_Inv2_RqSpd_Cval/1  "API2_Inv2_RqSpd_Cval"
  pneAux_rebuild_generic_std_sf/53 -> aOverVoltPrim_Stat_SATP/1  "aOverVoltPrim_Stat_SATP"
  pneAux_rebuild_generic_std_sf/52 -> AmbWarn_Rq_Trlr5/1  "AmbWarn_Rq_Trlr5"
  pneAux_rebuild_generic_std_sf/51 -> AmbWarn_Rq_Trlr4/1  "AmbWarn_Rq_Trlr4"
  pneAux_rebuild_generic_std_sf/50 -> AmbWarn_Rq_Trlr3/1  "AmbWarn_Rq_Trlr3"
  pneAux_rebuild_generic_std_sf/49 -> AmbWarn_Rq_Trlr2/1  "AmbWarn_Rq_Trlr2"
  pneAux_rebuild_generic_std_sf/48 -> AmbWarn_Rq_Trlr/1  "AmbWarn_Rq_Trlr"
  pneAux_rebuild_generic_std_sf/47 -> AirComp_Stat_SATP/1  "AirComp_Stat_SATP"
  pneAux_rebuild_generic_std_sf/46 -> aImplsblMdCmdErr_Stat_SATP/1  "aImplsblMdCmdErr_Stat_SATP"
  pneAux_rebuild_generic_std_sf/45 -> aBrkAirPress2_Stat_SATP/1  "aBrkAirPress2_Stat_SATP"
  pneAux_rebuild_generic_std_sf/44 -> aBrkAirPress2_Cval_SATP/1  "aBrkAirPress2_Cval_SATP"
  pneAux_rebuild_generic_std_sf/43 -> aBrkAirPress1_Stat_SATP/1  "aBrkAirPress1_Stat_SATP"
  pneAux_rebuild_generic_std_sf/42 -> aBrkAirPress1_Cval_SATP/1  "aBrkAirPress1_Cval_SATP"
  pneAux_rebuild_generic_std_sf/41 -> aAutoOpMd_Stat_SATP/1  "aAutoOpMd_Stat_SATP"
  pneAux_rebuild_generic_std_sf/40 -> aAutoMd3To1Rdy_Stat_SATP/1  "aAutoMd3To1Rdy_Stat_SATP"
  pneAux_rebuild_generic_std_sf/39 -> aAutoMd1To3Rdy_Stat_SATP/1  "aAutoMd1To3Rdy_Stat_SATP"
  pneAux_rebuild_generic_std_sf/38 -> aAutoMd1To2Rdy_Stat_SATP/1  "aAutoMd1To2Rdy_Stat_SATP"
  pneAux_rebuild_generic_std_sf/37 -> aAirComp_Stat_SATP/1  "aAirComp_Stat_SATP"
  pneAux_rebuild_generic_std_sf/36 -> pneAux_trailerAxle3_right_stABSOutValve/1  "pneAux_trailerAxle3_right_stABSOutValve"
  pneAux_rebuild_generic_std_sf/35 -> pneAux_trailerAxle3_right_stABSInValve/1  "pneAux_trailerAxle3_right_stABSInValve"
  pneAux_rebuild_generic_std_sf/34 -> pneAux_trailerAxle3_load/1  "pneAux_trailerAxle3_load"
  pneAux_rebuild_generic_std_sf/33 -> pneAux_trailerAxle3_left_stABSOutValve/1  "pneAux_trailerAxle3_left_stABSOutValve"
  pneAux_rebuild_generic_std_sf/32 -> pneAux_trailerAxle3_left_stABSInValve/1  "pneAux_trailerAxle3_left_stABSInValve"
  pneAux_rebuild_generic_std_sf/31 -> pneAux_trailerAxle2_right_stABSOutValve/1  "pneAux_trailerAxle2_right_stABSOutValve"
  pneAux_rebuild_generic_std_sf/30 -> pneAux_trailerAxle2_right_stABSInValve/1  "pneAux_trailerAxle2_right_stABSInValve"
  pneAux_rebuild_generic_std_sf/29 -> pneAux_trailerAxle2_load/1  "pneAux_trailerAxle2_load"
  pneAux_rebuild_generic_std_sf/28 -> pneAux_trailerAxle2_left_stABSOutValve/1  "pneAux_trailerAxle2_left_stABSOutValve"
  pneAux_rebuild_generic_std_sf/27 -> pneAux_trailerAxle2_left_stABSInValve/1  "pneAux_trailerAxle2_left_stABSInValve"
  pneAux_rebuild_generic_std_sf/26 -> pneAux_trailerAxle1_right_stABSOutValve/1  "pneAux_trailerAxle1_right_stABSOutValve"
  pneAux_rebuild_generic_std_sf/25 -> pneAux_trailerAxle1_right_stABSInValve/1  "pneAux_trailerAxle1_right_stABSInValve"
  pneAux_rebuild_generic_std_sf/24 -> pneAux_trailerAxle1_load/1  "pneAux_trailerAxle1_load"
  pneAux_rebuild_generic_std_sf/23 -> pneAux_trailerAxle1_left_stABSOutValve/1  "pneAux_trailerAxle1_left_stABSOutValve"
  pneAux_rebuild_generic_std_sf/22 -> pneAux_trailerAxle1_left_stABSInValve/1  "pneAux_trailerAxle1_left_stABSInValve"
  pneAux_rebuild_generic_std_sf/21 -> pneAux_TCV_pDmd_Rear_Right/1  "pneAux_TCV_pDmd_Rear_Right"
  pneAux_rebuild_generic_std_sf/20 -> pneAux_TCV_pDmd_Rear_Left/1  "pneAux_TCV_pDmd_Rear_Left"
  pneAux_rebuild_generic_std_sf/19 -> pneAux_TCV_pDmd_Front_Right/1  "pneAux_TCV_pDmd_Front_Right"
  pneAux_rebuild_generic_std_sf/18 -> pneAux_TCV_pDmd_Front_Left/1  "pneAux_TCV_pDmd_Front_Left"
  pneAux_rebuild_generic_std_sf/17 -> pneAux_pSollPkBrk/1  "pneAux_pSollPkBrk"
  pneAux_rebuild_generic_std_sf/16 -> pneAux_pSoll_TCV_p43/1  "pneAux_pSoll_TCV_p43"
  pneAux_rebuild_generic_std_sf/15 -> pneAux_EAPU_overrun/1  "pneAux_EAPU_overrun"
  pneAux_rebuild_generic_std_sf/14 -> pneAux_Drs_Rq/1  "pneAux_Drs_Rq"
  pneAux_rebuild_generic_std_sf/13 -> pneAux_Axle4_load/1  "pneAux_Axle4_load"
  pneAux_rebuild_generic_std_sf/12 -> pneAux_Axle3_load/1  "pneAux_Axle3_load"
  pneAux_rebuild_generic_std_sf/11 -> pneAux_Axle2_load/1  "pneAux_Axle2_load"
  pneAux_rebuild_generic_std_sf/10 -> pneAux_Axle1_load/1  "pneAux_Axle1_load"
  pneAux_rebuild_generic_std_sf/9 -> pneAux_A3_Ri_Rq/1  "pneAux_A3_Ri_Rq"
  pneAux_rebuild_generic_std_sf/8 -> pneAux_A3_LoLi_Rq/1  "pneAux_A3_LoLi_Rq"
  pneAux_rebuild_generic_std_sf/7 -> pneAux_A3_Le_Rq/1  "pneAux_A3_Le_Rq"
  pneAux_rebuild_generic_std_sf/6 -> pneAux_A2_Ri_Rq/1  "pneAux_A2_Ri_Rq"
  pneAux_rebuild_generic_std_sf/5 -> pneAux_A2_LoLi_Rq/1  "pneAux_A2_LoLi_Rq"
  pneAux_rebuild_generic_std_sf/4 -> pneAux_A2_Le_Rq/1  "pneAux_A2_Le_Rq"
  pneAux_rebuild_generic_std_sf/3 -> pneAux_A1_Ri_Rq/1  "pneAux_A1_Ri_Rq"
  pneAux_rebuild_generic_std_sf/2 -> pneAux_A1_LoLi_Rq/1  "pneAux_A1_LoLi_Rq"
  pneAux_rebuild_generic_std_sf/1 -> pneAux_A1_Le_Rq/1  "pneAux_A1_Le_Rq"
  pne_susp_A3_Ri_Posn/1 -> pneAux_rebuild_generic_std_sf/67  "pne_susp_A3_Ri_Posn"
  pne_susp_A3_Le_Posn/1 -> pneAux_rebuild_generic_std_sf/66  "pne_susp_A3_Le_Posn"
  pne_susp_A2_Ri_Posn/1 -> pneAux_rebuild_generic_std_sf/65  "pne_susp_A2_Ri_Posn"
  pne_susp_A2_Le_Posn/1 -> pneAux_rebuild_generic_std_sf/64  "pne_susp_A2_Le_Posn"
  pne_susp_A1_Ri_Posn/1 -> pneAux_rebuild_generic_std_sf/63  "pne_susp_A1_Ri_Posn"
  pne_susp_A1_Le_Posn/1 -> pneAux_rebuild_generic_std_sf/62  "pne_susp_A1_Le_Posn"
  pne_brk_WetLvl_Cntr/1 -> pneAux_rebuild_generic_std_sf/61  "pne_brk_WetLvl_Cntr"
  pne_brk_VTrailer_pRel/1 -> pneAux_rebuild_generic_std_sf/60  "pne_brk_VTrailer_pRel"
  pne_brk_V7_pRel/1 -> pneAux_rebuild_generic_std_sf/59  "pne_brk_V7_pRel"
  pne_brk_V4_pRel/1 -> pneAux_rebuild_generic_std_sf/58  "pne_brk_V4_pRel"
  pne_brk_V2_pRel/1 -> pneAux_rebuild_generic_std_sf/57  "pne_brk_V2_pRel"
  pne_brk_V1_pRel/1 -> pneAux_rebuild_generic_std_sf/56  "pne_brk_V1_pRel"
  pne_brk_TrailerAxle3_torque_sns/1 -> pneAux_rebuild_generic_std_sf/55  "pne_brk_TrailerAxle3_torque_sns"
  pne_brk_TrailerAxle3_BrakingForce_at8p5bar/1 -> pneAux_rebuild_generic_std_sf/54  "pne_brk_TrailerAxle3_BrakingForce_at8p5bar"
  pne_brk_TrailerAxle2_torque_sns/1 -> pneAux_rebuild_generic_std_sf/53  "pne_brk_TrailerAxle2_torque_sns"
  pne_brk_TrailerAxle2_BrakingForce_at8p5bar/1 -> pneAux_rebuild_generic_std_sf/52  "pne_brk_TrailerAxle2_BrakingForce_at8p5bar"
  pne_brk_TrailerAxle1_torque_sns/1 -> pneAux_rebuild_generic_std_sf/51  "pne_brk_TrailerAxle1_torque_sns"
  pne_brk_TrailerAxle1_BrakingForce_at8p5bar/1 -> pneAux_rebuild_generic_std_sf/50  "pne_brk_TrailerAxle1_BrakingForce_at8p5bar"
  pne_brk_Trailer_RV_Rear_pAct/1 -> pneAux_rebuild_generic_std_sf/49  "pne_brk_Trailer_RV_Rear_pAct"
  pne_brk_Trailer_RV_Front_pAct/1 -> pneAux_rebuild_generic_std_sf/48  "pne_brk_Trailer_RV_Front_pAct"
  pne_brk_rotVel_t3r/1 -> pneAux_rebuild_generic_std_sf/47  "pne_brk_rotVel_t3r"
  pne_brk_rotVel_t3l/1 -> pneAux_rebuild_generic_std_sf/46  "pne_brk_rotVel_t3l"
  pne_brk_rotVel_t2r/1 -> pneAux_rebuild_generic_std_sf/45  "pne_brk_rotVel_t2r"
  pne_brk_rotVel_t2l/1 -> pneAux_rebuild_generic_std_sf/44  "pne_brk_rotVel_t2l"
  pne_brk_rotVel_t1r/1 -> pneAux_rebuild_generic_std_sf/43  "pne_brk_rotVel_t1r"
  pne_brk_rotVel_t1l/1 -> pneAux_rebuild_generic_std_sf/42  "pne_brk_rotVel_t1l"
  pne_brk_reg_active/1 -> pneAux_rebuild_generic_std_sf/41  "pne_brk_reg_active"
  pne_brk_pRelPkBrk/1 -> pneAux_rebuild_generic_std_sf/40  "pne_brk_pRelPkBrk"
  pne_brk_CompON/1 -> pneAux_rebuild_generic_std_sf/39  "pne_brk_CompON"
  pne_brk_BrkWearRA2Rt/1 -> pneAux_rebuild_generic_std_sf/38  "pne_brk_BrkWearRA2Rt"
  pne_brk_BrkWearRA2Lt/1 -> pneAux_rebuild_generic_std_sf/37  "pne_brk_BrkWearRA2Lt"
  pne_brk_BrkWearRA1Rt/1 -> pneAux_rebuild_generic_std_sf/36  "pne_brk_BrkWearRA1Rt"
  pne_brk_BrkWearRA1Lt/1 -> pneAux_rebuild_generic_std_sf/35  "pne_brk_BrkWearRA1Lt"
  pne_brk_BrkWearFA2Rt/1 -> pneAux_rebuild_generic_std_sf/34  "pne_brk_BrkWearFA2Rt"
  pne_brk_BrkWearFA2Lt/1 -> pneAux_rebuild_generic_std_sf/33  "pne_brk_BrkWearFA2Lt"
  pne_brk_BrkWearFA1Rt/1 -> pneAux_rebuild_generic_std_sf/32  "pne_brk_BrkWearFA1Rt"
  pne_brk_BrkWearFA1Lt/1 -> pneAux_rebuild_generic_std_sf/31  "pne_brk_BrkWearFA1Lt"
  pne_brk_BrkWearAARt/1 -> pneAux_rebuild_generic_std_sf/30  "pne_brk_BrkWearAARt"
  pne_brk_BrkWearAALt/1 -> pneAux_rebuild_generic_std_sf/29  "pne_brk_BrkWearAALt"
  pne_brk_Axle4_torque_sns/1 -> pneAux_rebuild_generic_std_sf/28  "pne_brk_Axle4_torque_sns"
  pne_brk_Axle3_torque_sns/1 -> pneAux_rebuild_generic_std_sf/27  "pne_brk_Axle3_torque_sns"
  pne_brk_Axle2_torque_sns/1 -> pneAux_rebuild_generic_std_sf/26  "pne_brk_Axle2_torque_sns"
  pne_brk_Axle1_torque_sns/1 -> pneAux_rebuild_generic_std_sf/25  "pne_brk_Axle1_torque_sns"
  mec_veh_transVel/1 -> pneAux_rebuild_generic_std_sf/24  "mec_veh_transVel"
  mec_veh_TrailerAxleLoad3/1 -> pneAux_rebuild_generic_std_sf/23  "mec_veh_TrailerAxleLoad3"
  mec_veh_TrailerAxleLoad2/1 -> pneAux_rebuild_generic_std_sf/22  "mec_veh_TrailerAxleLoad2"
  mec_veh_TrailerAxleLoad1/1 -> pneAux_rebuild_generic_std_sf/21  "mec_veh_TrailerAxleLoad1"
  mec_veh_AxleLoad4/1 -> pneAux_rebuild_generic_std_sf/20  "mec_veh_AxleLoad4"
  mec_veh_AxleLoad3/1 -> pneAux_rebuild_generic_std_sf/19  "mec_veh_AxleLoad3"
  mec_veh_AxleLoad2/1 -> pneAux_rebuild_generic_std_sf/18  "mec_veh_AxleLoad2"
  mec_veh_AxleLoad1/1 -> pneAux_rebuild_generic_std_sf/17  "mec_veh_AxleLoad1"
  hvs_InverterAirCompressor_hvVoltage/1 -> pneAux_rebuild_generic_std_sf/16  "hvs_InverterAirCompressor_hvVoltage"
  hvs_InverterAirCompressor_hvCurrent/1 -> pneAux_rebuild_generic_std_sf/15  "hvs_InverterAirCompressor_hvCurrent"
  hvs_AirCompressor_nEmot/1 -> pneAux_rebuild_generic_std_sf/14  "hvs_AirCompressor_nEmot"
  drv_PkBrkLever_pos/1 -> pneAux_rebuild_generic_std_sf/13  "drv_PkBrkLever_pos"
  drv_PkBrk/1 -> pneAux_rebuild_generic_std_sf/12  "drv_PkBrk"
  drv_Knl_Rq/1 -> pneAux_rebuild_generic_std_sf/11  "drv_Knl_Rq"
  drv_DrS_Rq/1 -> pneAux_rebuild_generic_std_sf/10  "drv_DrS_Rq"
  pne_MTBmodusSwAllowed/1 -> pneAux_rebuild_generic_std_sf/9  "pne_MTBmodusSwAllowed"
  EngRPM_Cval_CPC3/1 -> pneAux_rebuild_generic_std_sf/8  "EngRPM_Cval_CPC3"
  drv_Trlr_Air_Sup_Sw_Stat/1 -> pneAux_rebuild_generic_std_sf/7  "drv_Trlr_Air_Sup_Sw_Stat"
  drv_PB_Sw_Stat_SATP/1 -> pneAux_rebuild_generic_std_sf/6  "drv_PB_Sw_Stat_SATP"
  ch_Clutch_Stat_CPC/1 -> pneAux_rebuild_generic_std_sf/5  "ch_Clutch_Stat_CPC"
  BS_PB_Fct_Rq/1 -> pneAux_rebuild_generic_std_sf/4  "BS_PB_Fct_Rq"
  aSatpAutoOpMd_Cmd_SDS/1 -> pneAux_rebuild_generic_std_sf/3  "aSatpAutoOpMd_Cmd_SDS"
  ActlEngPctTrq_Cval/1 -> pneAux_rebuild_generic_std_sf/2  "ActlEngPctTrq_Cval"
  env_Temperature/1 -> pneAux_rebuild_generic_std_sf/1  "env_Temperature"
